simulink model "model"  (R2014a)
(part 2 of 3)

  _CN_171253574_150000_CN_129055610_150000 : powerlib/Elements/Distributed Parameters Line  Phases=3  Frequency=60  Resistance=[0.01273 0.3864]  Inductance="[0.9337e-3  4.1264e-3]"  Capacitance=[12.74e-9 7.751e-9]  Length=23.0398  x1=[0 0 0 0; 0.0001244 0 0 0; 0.0002488 0 0 0; 0.0003733 0 0 0; 0.0004977 0 0 0; 0.0006221 0 0 0]  x2=[0 0 0 0; 0.0001244 0 0 0; 0.0002488 0 0 0; 0.0003733 0 0 0; 0.0004977 0 0 0; 0.0006221 0 0 0]  x3=[0 0 0 0; 0.0001244 0 0 0; 0.0002488 0 0 0; 0.0003733 0 0 0; 0.0004977 0 0 0; 0.0006221 0 0 0]  x4=[0 0 0 0; 0.0001244 0 0 0; 0.0002488 0 0 0; 0.0003733 0 0 0; 0.0004977 0 0 0; 0.0006221 0 0 0]  x5=0  V1=ones(3,3)  V2=ones(3,3)  I1=ones(3,3)  I2=ones(3,3)  nHarmo=1  Measurements=None
  _CN_171253574_150000_CN_163226993_150000 : powerlib/Elements/Distributed Parameters Line  Phases=3  Frequency=60  Resistance=[0.01273 0.3864]  Inductance="[0.9337e-3  4.1264e-3]"  Capacitance=[12.74e-9 7.751e-9]  Length=4.3634  x1=[0 0 0 0; 0.0001244 0 0 0; 0.0002488 0 0 0; 0.0003733 0 0 0; 0.0004977 0 0 0; 0.0006221 0 0 0]  x2=[0 0 0 0; 0.0001244 0 0 0; 0.0002488 0 0 0; 0.0003733 0 0 0; 0.0004977 0 0 0; 0.0006221 0 0 0]  x3=[0 0 0 0; 0.0001244 0 0 0; 0.0002488 0 0 0; 0.0003733 0 0 0; 0.0004977 0 0 0; 0.0006221 0 0 0]  x4=[0 0 0 0; 0.0001244 0 0 0; 0.0002488 0 0 0; 0.0003733 0 0 0; 0.0004977 0 0 0; 0.0006221 0 0 0]  x5=0  V1=ones(3,3)  V2=ones(3,3)  I1=ones(3,3)  I2=ones(3,3)  nHarmo=1  Measurements=None
  _CN_183668286_220000_CN_151168335_220000 : powerlib/Elements/Distributed Parameters Line  Phases=3  Frequency=60  Resistance=[0.01273 0.3864]  Inductance="[0.9337e-3  4.1264e-3]"  Capacitance=[12.74e-9 7.751e-9]  Length=7.5354  x1=[0 0 0 0; 0.0001244 0 0 0; 0.0002488 0 0 0; 0.0003733 0 0 0; 0.0004977 0 0 0; 0.0006221 0 0 0]  x2=[0 0 0 0; 0.0001244 0 0 0; 0.0002488 0 0 0; 0.0003733 0 0 0; 0.0004977 0 0 0; 0.0006221 0 0 0]  x3=[0 0 0 0; 0.0001244 0 0 0; 0.0002488 0 0 0; 0.0003733 0 0 0; 0.0004977 0 0 0; 0.0006221 0 0 0]  x4=[0 0 0 0; 0.0001244 0 0 0; 0.0002488 0 0 0; 0.0003733 0 0 0; 0.0004977 0 0 0; 0.0006221 0 0 0]  x5=0  V1=ones(3,3)  V2=ones(3,3)  I1=ones(3,3)  I2=ones(3,3)  nHarmo=1  Measurements=None
  _CN_24636044_150000_CN_402947133_150000 : powerlib/Elements/Distributed Parameters Line  Phases=3  Frequency=60  Resistance=[0.01273 0.3864]  Inductance="[0.9337e-3  4.1264e-3]"  Capacitance=[12.74e-9 7.751e-9]  Length=13.2604  x1=[0 0 0 0; 0.0001244 0 0 0; 0.0002488 0 0 0; 0.0003733 0 0 0; 0.0004977 0 0 0; 0.0006221 0 0 0]  x2=[0 0 0 0; 0.0001244 0 0 0; 0.0002488 0 0 0; 0.0003733 0 0 0; 0.0004977 0 0 0; 0.0006221 0 0 0]  x3=[0 0 0 0; 0.0001244 0 0 0; 0.0002488 0 0 0; 0.0003733 0 0 0; 0.0004977 0 0 0; 0.0006221 0 0 0]  x4=[0 0 0 0; 0.0001244 0 0 0; 0.0002488 0 0 0; 0.0003733 0 0 0; 0.0004977 0 0 0; 0.0006221 0 0 0]  x5=0  V1=ones(3,3)  V2=ones(3,3)  I1=ones(3,3)  I2=ones(3,3)  nHarmo=1  Measurements=None
  _CN_24636044_220000_CN_131715746_220000 : powerlib/Elements/Distributed Parameters Line  Phases=3  Frequency=60  Resistance=[0.01273 0.3864]  Inductance="[0.9337e-3  4.1264e-3]"  Capacitance=[12.74e-9 7.751e-9]  Length=90.51  x1=[0 0 0 0; 0.0001244 0 0 0; 0.0002488 0 0 0; 0.0003733 0 0 0; 0.0004977 0 0 0; 0.0006221 0 0 0]  x2=[0 0 0 0; 0.0001244 0 0 0; 0.0002488 0 0 0; 0.0003733 0 0 0; 0.0004977 0 0 0; 0.0006221 0 0 0]  x3=[0 0 0 0; 0.0001244 0 0 0; 0.0002488 0 0 0; 0.0003733 0 0 0; 0.0004977 0 0 0; 0.0006221 0 0 0]  x4=[0 0 0 0; 0.0001244 0 0 0; 0.0002488 0 0 0; 0.0003733 0 0 0; 0.0004977 0 0 0; 0.0006221 0 0 0]  x5=0  V1=ones(3,3)  V2=ones(3,3)  I1=ones(3,3)  I2=ones(3,3)  nHarmo=1  Measurements=None
  _CN_24636044_220000_CN_144651478_220000 : powerlib/Elements/Distributed Parameters Line  Phases=3  Frequency=60  Resistance=[0.01273 0.3864]  Inductance="[0.9337e-3  4.1264e-3]"  Capacitance=[12.74e-9 7.751e-9]  Length=28.1072  x1=[0 0 0 0; 0.0001244 0 0 0; 0.0002488 0 0 0; 0.0003733 0 0 0; 0.0004977 0 0 0; 0.0006221 0 0 0]  x2=[0 0 0 0; 0.0001244 0 0 0; 0.0002488 0 0 0; 0.0003733 0 0 0; 0.0004977 0 0 0; 0.0006221 0 0 0]  x3=[0 0 0 0; 0.0001244 0 0 0; 0.0002488 0 0 0; 0.0003733 0 0 0; 0.0004977 0 0 0; 0.0006221 0 0 0]  x4=[0 0 0 0; 0.0001244 0 0 0; 0.0002488 0 0 0; 0.0003733 0 0 0; 0.0004977 0 0 0; 0.0006221 0 0 0]  x5=0  V1=ones(3,3)  V2=ones(3,3)  I1=ones(3,3)  I2=ones(3,3)  nHarmo=1  Measurements=None
  _CN_24636044_220000_CN_144654759_220000 : powerlib/Elements/Distributed Parameters Line  Phases=3  Frequency=60  Resistance=[0.01273 0.3864]  Inductance="[0.9337e-3  4.1264e-3]"  Capacitance=[12.74e-9 7.751e-9]  Length=18.5067  x1=[0 0 0 0; 0.0001244 0 0 0; 0.0002488 0 0 0; 0.0003733 0 0 0; 0.0004977 0 0 0; 0.0006221 0 0 0]  x2=[0 0 0 0; 0.0001244 0 0 0; 0.0002488 0 0 0; 0.0003733 0 0 0; 0.0004977 0 0 0; 0.0006221 0 0 0]  x3=[0 0 0 0; 0.0001244 0 0 0; 0.0002488 0 0 0; 0.0003733 0 0 0; 0.0004977 0 0 0; 0.0006221 0 0 0]  x4=[0 0 0 0; 0.0001244 0 0 0; 0.0002488 0 0 0; 0.0003733 0 0 0; 0.0004977 0 0 0; 0.0006221 0 0 0]  x5=0  V1=ones(3,3)  V2=ones(3,3)  I1=ones(3,3)  I2=ones(3,3)  nHarmo=1  Measurements=None
  _CN_24636044_220000_CN_144762180_220000 : powerlib/Elements/Distributed Parameters Line  Phases=3  Frequency=60  Resistance=[0.01273 0.3864]  Inductance="[0.9337e-3  4.1264e-3]"  Capacitance=[12.74e-9 7.751e-9]  Length=13.8029  x1=[0 0 0 0; 0.0001244 0 0 0; 0.0002488 0 0 0; 0.0003733 0 0 0; 0.0004977 0 0 0; 0.0006221 0 0 0]  x2=[0 0 0 0; 0.0001244 0 0 0; 0.0002488 0 0 0; 0.0003733 0 0 0; 0.0004977 0 0 0; 0.0006221 0 0 0]  x3=[0 0 0 0; 0.0001244 0 0 0; 0.0002488 0 0 0; 0.0003733 0 0 0; 0.0004977 0 0 0; 0.0006221 0 0 0]  x4=[0 0 0 0; 0.0001244 0 0 0; 0.0002488 0 0 0; 0.0003733 0 0 0; 0.0004977 0 0 0; 0.0006221 0 0 0]  x5=0  V1=ones(3,3)  V2=ones(3,3)  I1=ones(3,3)  I2=ones(3,3)  nHarmo=1  Measurements=None
  _CN_24636044_220000_CN_151166980_220000 : powerlib/Elements/Distributed Parameters Line  Phases=3  Frequency=60  Resistance=[0.01273 0.3864]  Inductance="[0.9337e-3  4.1264e-3]"  Capacitance=[12.74e-9 7.751e-9]  Length=57.0251  x1=[0 0 0 0; 0.0001244 0 0 0; 0.0002488 0 0 0; 0.0003733 0 0 0; 0.0004977 0 0 0; 0.0006221 0 0 0]  x2=[0 0 0 0; 0.0001244 0 0 0; 0.0002488 0 0 0; 0.0003733 0 0 0; 0.0004977 0 0 0; 0.0006221 0 0 0]  x3=[0 0 0 0; 0.0001244 0 0 0; 0.0002488 0 0 0; 0.0003733 0 0 0; 0.0004977 0 0 0; 0.0006221 0 0 0]  x4=[0 0 0 0; 0.0001244 0 0 0; 0.0002488 0 0 0; 0.0003733 0 0 0; 0.0004977 0 0 0; 0.0006221 0 0 0]  x5=0  V1=ones(3,3)  V2=ones(3,3)  I1=ones(3,3)  I2=ones(3,3)  nHarmo=1  Measurements=None
  _CN_24636044_220000_CN_151168335_220000 : powerlib/Elements/Distributed Parameters Line  Phases=3  Frequency=60  Resistance=[0.01273 0.3864]  Inductance="[0.9337e-3  4.1264e-3]"  Capacitance=[12.74e-9 7.751e-9]  Length=19.5147  x1=[0 0 0 0; 0.0001244 0 0 0; 0.0002488 0 0 0; 0.0003733 0 0 0; 0.0004977 0 0 0; 0.0006221 0 0 0]  x2=[0 0 0 0; 0.0001244 0 0 0; 0.0002488 0 0 0; 0.0003733 0 0 0; 0.0004977 0 0 0; 0.0006221 0 0 0]  x3=[0 0 0 0; 0.0001244 0 0 0; 0.0002488 0 0 0; 0.0003733 0 0 0; 0.0004977 0 0 0; 0.0006221 0 0 0]  x4=[0 0 0 0; 0.0001244 0 0 0; 0.0002488 0 0 0; 0.0003733 0 0 0; 0.0004977 0 0 0; 0.0006221 0 0 0]  x5=0  V1=ones(3,3)  V2=ones(3,3)  I1=ones(3,3)  I2=ones(3,3)  nHarmo=1  Measurements=None
  _CN_24636044_220000_CN_24636062_220000 : powerlib/Elements/Distributed Parameters Line  Phases=3  Frequency=60  Resistance=[0.01273 0.3864]  Inductance="[0.9337e-3  4.1264e-3]"  Capacitance=[12.74e-9 7.751e-9]  Length=15.5637  x1=[0 0 0 0; 0.0001244 0 0 0; 0.0002488 0 0 0; 0.0003733 0 0 0; 0.0004977 0 0 0; 0.0006221 0 0 0]  x2=[0 0 0 0; 0.0001244 0 0 0; 0.0002488 0 0 0; 0.0003733 0 0 0; 0.0004977 0 0 0; 0.0006221 0 0 0]  x3=[0 0 0 0; 0.0001244 0 0 0; 0.0002488 0 0 0; 0.0003733 0 0 0; 0.0004977 0 0 0; 0.0006221 0 0 0]  x4=[0 0 0 0; 0.0001244 0 0 0; 0.0002488 0 0 0; 0.0003733 0 0 0; 0.0004977 0 0 0; 0.0006221 0 0 0]  x5=0  V1=ones(3,3)  V2=ones(3,3)  I1=ones(3,3)  I2=ones(3,3)  nHarmo=1  Measurements=None
  _CN_24636044_220000_CN_435865807_220000 : powerlib/Elements/Distributed Parameters Line  Phases=3  Frequency=60  Resistance=[0.01273 0.3864]  Inductance="[0.9337e-3  4.1264e-3]"  Capacitance=[12.74e-9 7.751e-9]  Length=24.8935  x1=[0 0 0 0; 0.0001244 0 0 0; 0.0002488 0 0 0; 0.0003733 0 0 0; 0.0004977 0 0 0; 0.0006221 0 0 0]  x2=[0 0 0 0; 0.0001244 0 0 0; 0.0002488 0 0 0; 0.0003733 0 0 0; 0.0004977 0 0 0; 0.0006221 0 0 0]  x3=[0 0 0 0; 0.0001244 0 0 0; 0.0002488 0 0 0; 0.0003733 0 0 0; 0.0004977 0 0 0; 0.0006221 0 0 0]  x4=[0 0 0 0; 0.0001244 0 0 0; 0.0002488 0 0 0; 0.0003733 0 0 0; 0.0004977 0 0 0; 0.0006221 0 0 0]  x5=0  V1=ones(3,3)  V2=ones(3,3)  I1=ones(3,3)  I2=ones(3,3)  nHarmo=1  Measurements=None
  _CN_24636044_400000_CN_129055610_400000 : powerlib/Elements/Distributed Parameters Line  Phases=3  Frequency=60  Resistance=[0.01273 0.3864]  Inductance="[0.9337e-3  4.1264e-3]"  Capacitance=[12.74e-9 7.751e-9]  Length=68.1978  x1=[0 0 0 0; 0.0001244 0 0 0; 0.0002488 0 0 0; 0.0003733 0 0 0; 0.0004977 0 0 0; 0.0006221 0 0 0]  x2=[0 0 0 0; 0.0001244 0 0 0; 0.0002488 0 0 0; 0.0003733 0 0 0; 0.0004977 0 0 0; 0.0006221 0 0 0]  x3=[0 0 0 0; 0.0001244 0 0 0; 0.0002488 0 0 0; 0.0003733 0 0 0; 0.0004977 0 0 0; 0.0006221 0 0 0]  x4=[0 0 0 0; 0.0001244 0 0 0; 0.0002488 0 0 0; 0.0003733 0 0 0; 0.0004977 0 0 0; 0.0006221 0 0 0]  x5=0  V1=ones(3,3)  V2=ones(3,3)  I1=ones(3,3)  I2=ones(3,3)  nHarmo=1  Measurements=None
  _CN_24636044_400000_CN_131715746_400000 : powerlib/Elements/Distributed Parameters Line  Phases=3  Frequency=60  Resistance=[0.01273 0.3864]  Inductance="[0.9337e-3  4.1264e-3]"  Capacitance=[12.74e-9 7.751e-9]  Length=53.1895  x1=[0 0 0 0; 0.0001244 0 0 0; 0.0002488 0 0 0; 0.0003733 0 0 0; 0.0004977 0 0 0; 0.0006221 0 0 0]  x2=[0 0 0 0; 0.0001244 0 0 0; 0.0002488 0 0 0; 0.0003733 0 0 0; 0.0004977 0 0 0; 0.0006221 0 0 0]  x3=[0 0 0 0; 0.0001244 0 0 0; 0.0002488 0 0 0; 0.0003733 0 0 0; 0.0004977 0 0 0; 0.0006221 0 0 0]  x4=[0 0 0 0; 0.0001244 0 0 0; 0.0002488 0 0 0; 0.0003733 0 0 0; 0.0004977 0 0 0; 0.0006221 0 0 0]  x5=0  V1=ones(3,3)  V2=ones(3,3)  I1=ones(3,3)  I2=ones(3,3)  nHarmo=1  Measurements=None
  _CN_24636044_400000_CN_144608818_400000 : powerlib/Elements/Distributed Parameters Line  Phases=3  Frequency=60  Resistance=[0.01273 0.3864]  Inductance="[0.9337e-3  4.1264e-3]"  Capacitance=[12.74e-9 7.751e-9]  Length=25.0456  x1=[0 0 0 0; 0.0001244 0 0 0; 0.0002488 0 0 0; 0.0003733 0 0 0; 0.0004977 0 0 0; 0.0006221 0 0 0]  x2=[0 0 0 0; 0.0001244 0 0 0; 0.0002488 0 0 0; 0.0003733 0 0 0; 0.0004977 0 0 0; 0.0006221 0 0 0]  x3=[0 0 0 0; 0.0001244 0 0 0; 0.0002488 0 0 0; 0.0003733 0 0 0; 0.0004977 0 0 0; 0.0006221 0 0 0]  x4=[0 0 0 0; 0.0001244 0 0 0; 0.0002488 0 0 0; 0.0003733 0 0 0; 0.0004977 0 0 0; 0.0006221 0 0 0]  x5=0  V1=ones(3,3)  V2=ones(3,3)  I1=ones(3,3)  I2=ones(3,3)  nHarmo=1  Measurements=None
  _CN_24636044_400000_CN_151168335_400000 : powerlib/Elements/Distributed Parameters Line  Phases=3  Frequency=60  Resistance=[0.01273 0.3864]  Inductance="[0.9337e-3  4.1264e-3]"  Capacitance=[12.74e-9 7.751e-9]  Length=18.3774  x1=[0 0 0 0; 0.0001244 0 0 0; 0.0002488 0 0 0; 0.0003733 0 0 0; 0.0004977 0 0 0; 0.0006221 0 0 0]  x2=[0 0 0 0; 0.0001244 0 0 0; 0.0002488 0 0 0; 0.0003733 0 0 0; 0.0004977 0 0 0; 0.0006221 0 0 0]  x3=[0 0 0 0; 0.0001244 0 0 0; 0.0002488 0 0 0; 0.0003733 0 0 0; 0.0004977 0 0 0; 0.0006221 0 0 0]  x4=[0 0 0 0; 0.0001244 0 0 0; 0.0002488 0 0 0; 0.0003733 0 0 0; 0.0004977 0 0 0; 0.0006221 0 0 0]  x5=0  V1=ones(3,3)  V2=ones(3,3)  I1=ones(3,3)  I2=ones(3,3)  nHarmo=1  Measurements=None
  _CN_24636062_220000_CN_183668286_220000 : powerlib/Elements/Distributed Parameters Line  Phases=3  Frequency=60  Resistance=[0.01273 0.3864]  Inductance="[0.9337e-3  4.1264e-3]"  Capacitance=[12.74e-9 7.751e-9]  Length=4.494  x1=[0 0 0 0; 0.0001244 0 0 0; 0.0002488 0 0 0; 0.0003733 0 0 0; 0.0004977 0 0 0; 0.0006221 0 0 0]  x2=[0 0 0 0; 0.0001244 0 0 0; 0.0002488 0 0 0; 0.0003733 0 0 0; 0.0004977 0 0 0; 0.0006221 0 0 0]  x3=[0 0 0 0; 0.0001244 0 0 0; 0.0002488 0 0 0; 0.0003733 0 0 0; 0.0004977 0 0 0; 0.0006221 0 0 0]  x4=[0 0 0 0; 0.0001244 0 0 0; 0.0002488 0 0 0; 0.0003733 0 0 0; 0.0004977 0 0 0; 0.0006221 0 0 0]  x5=0  V1=ones(3,3)  V2=ones(3,3)  I1=ones(3,3)  I2=ones(3,3)  nHarmo=1  Measurements=None
  _CN_402947133_220000_CN_144762180_220000 : powerlib/Elements/Distributed Parameters Line  Phases=3  Frequency=60  Resistance=[0.01273 0.3864]  Inductance="[0.9337e-3  4.1264e-3]"  Capacitance=[12.74e-9 7.751e-9]  Length=1.5227  x1=[0 0 0 0; 0.0001244 0 0 0; 0.0002488 0 0 0; 0.0003733 0 0 0; 0.0004977 0 0 0; 0.0006221 0 0 0]  x2=[0 0 0 0; 0.0001244 0 0 0; 0.0002488 0 0 0; 0.0003733 0 0 0; 0.0004977 0 0 0; 0.0006221 0 0 0]  x3=[0 0 0 0; 0.0001244 0 0 0; 0.0002488 0 0 0; 0.0003733 0 0 0; 0.0004977 0 0 0; 0.0006221 0 0 0]  x4=[0 0 0 0; 0.0001244 0 0 0; 0.0002488 0 0 0; 0.0003733 0 0 0; 0.0004977 0 0 0; 0.0006221 0 0 0]  x5=0  V1=ones(3,3)  V2=ones(3,3)  I1=ones(3,3)  I2=ones(3,3)  nHarmo=1  Measurements=None
  _CN_435865807_220000_CN_131715746_220000 : powerlib/Elements/Distributed Parameters Line  Phases=3  Frequency=60  Resistance=[0.01273 0.3864]  Inductance="[0.9337e-3  4.1264e-3]"  Capacitance=[12.74e-9 7.751e-9]  Length=38.8013  x1=[0 0 0 0; 0.0001244 0 0 0; 0.0002488 0 0 0; 0.0003733 0 0 0; 0.0004977 0 0 0; 0.0006221 0 0 0]  x2=[0 0 0 0; 0.0001244 0 0 0; 0.0002488 0 0 0; 0.0003733 0 0 0; 0.0004977 0 0 0; 0.0006221 0 0 0]  x3=[0 0 0 0; 0.0001244 0 0 0; 0.0002488 0 0 0; 0.0003733 0 0 0; 0.0004977 0 0 0; 0.0006221 0 0 0]  x4=[0 0 0 0; 0.0001244 0 0 0; 0.0002488 0 0 0; 0.0003733 0 0 0; 0.0004977 0 0 0; 0.0006221 0 0 0]  x5=0  V1=ones(3,3)  V2=ones(3,3)  I1=ones(3,3)  I2=ones(3,3)  nHarmo=1  Measurements=None
  _CN_435865807_220000_CN_144596347_220000 : powerlib/Elements/Distributed Parameters Line  Phases=3  Frequency=60  Resistance=[0.01273 0.3864]  Inductance="[0.9337e-3  4.1264e-3]"  Capacitance=[12.74e-9 7.751e-9]  Length=34.808  x1=[0 0 0 0; 0.0001244 0 0 0; 0.0002488 0 0 0; 0.0003733 0 0 0; 0.0004977 0 0 0; 0.0006221 0 0 0]  x2=[0 0 0 0; 0.0001244 0 0 0; 0.0002488 0 0 0; 0.0003733 0 0 0; 0.0004977 0 0 0; 0.0006221 0 0 0]  x3=[0 0 0 0; 0.0001244 0 0 0; 0.0002488 0 0 0; 0.0003733 0 0 0; 0.0004977 0 0 0; 0.0006221 0 0 0]  x4=[0 0 0 0; 0.0001244 0 0 0; 0.0002488 0 0 0; 0.0003733 0 0 0; 0.0004977 0 0 0; 0.0006221 0 0 0]  x5=0  V1=ones(3,3)  V2=ones(3,3)  I1=ones(3,3)  I2=ones(3,3)  nHarmo=1  Measurements=None
  _CN_435865807_220000_CN_144703168_220000 : powerlib/Elements/Distributed Parameters Line  Phases=3  Frequency=60  Resistance=[0.01273 0.3864]  Inductance="[0.9337e-3  4.1264e-3]"  Capacitance=[12.74e-9 7.751e-9]  Length=56.7538  x1=[0 0 0 0; 0.0001244 0 0 0; 0.0002488 0 0 0; 0.0003733 0 0 0; 0.0004977 0 0 0; 0.0006221 0 0 0]  x2=[0 0 0 0; 0.0001244 0 0 0; 0.0002488 0 0 0; 0.0003733 0 0 0; 0.0004977 0 0 0; 0.0006221 0 0 0]  x3=[0 0 0 0; 0.0001244 0 0 0; 0.0002488 0 0 0; 0.0003733 0 0 0; 0.0004977 0 0 0; 0.0006221 0 0 0]  x4=[0 0 0 0; 0.0001244 0 0 0; 0.0002488 0 0 0; 0.0003733 0 0 0; 0.0004977 0 0 0; 0.0006221 0 0 0]  x5=0  V1=ones(3,3)  V2=ones(3,3)  I1=ones(3,3)  I2=ones(3,3)  nHarmo=1  Measurements=None
  _CN_47895778_220000_CN_127205502_220000 : powerlib/Elements/Distributed Parameters Line  Phases=3  Frequency=60  Resistance=[0.01273 0.3864]  Inductance="[0.9337e-3  4.1264e-3]"  Capacitance=[12.74e-9 7.751e-9]  Length=41.7466  x1=[0 0 0 0; 0.0001244 0 0 0; 0.0002488 0 0 0; 0.0003733 0 0 0; 0.0004977 0 0 0; 0.0006221 0 0 0]  x2=[0 0 0 0; 0.0001244 0 0 0; 0.0002488 0 0 0; 0.0003733 0 0 0; 0.0004977 0 0 0; 0.0006221 0 0 0]  x3=[0 0 0 0; 0.0001244 0 0 0; 0.0002488 0 0 0; 0.0003733 0 0 0; 0.0004977 0 0 0; 0.0006221 0 0 0]  x4=[0 0 0 0; 0.0001244 0 0 0; 0.0002488 0 0 0; 0.0003733 0 0 0; 0.0004977 0 0 0; 0.0006221 0 0 0]  x5=0  V1=ones(3,3)  V2=ones(3,3)  I1=ones(3,3)  I2=ones(3,3)  nHarmo=1  Measurements=None
  _CN_47911346_220000_CN_47895778_220000 : powerlib/Elements/Distributed Parameters Line  Phases=3  Frequency=60  Resistance=[0.01273 0.3864]  Inductance="[0.9337e-3  4.1264e-3]"  Capacitance=[12.74e-9 7.751e-9]  Length=0.71591  x1=[0 0 0 0; 0.0001244 0 0 0; 0.0002488 0 0 0; 0.0003733 0 0 0; 0.0004977 0 0 0; 0.0006221 0 0 0]  x2=[0 0 0 0; 0.0001244 0 0 0; 0.0002488 0 0 0; 0.0003733 0 0 0; 0.0004977 0 0 0; 0.0006221 0 0 0]  x3=[0 0 0 0; 0.0001244 0 0 0; 0.0002488 0 0 0; 0.0003733 0 0 0; 0.0004977 0 0 0; 0.0006221 0 0 0]  x4=[0 0 0 0; 0.0001244 0 0 0; 0.0002488 0 0 0; 0.0003733 0 0 0; 0.0004977 0 0 0; 0.0006221 0 0 0]  x5=0  V1=ones(3,3)  V2=ones(3,3)  I1=ones(3,3)  I2=ones(3,3)  nHarmo=1  Measurements=None
  _CN_47911346_400000_CN_144327157_400000 : powerlib/Elements/Distributed Parameters Line  Phases=3  Frequency=60  Resistance=[0.01273 0.3864]  Inductance="[0.9337e-3  4.1264e-3]"  Capacitance=[12.74e-9 7.751e-9]  Length=17.6368  x1=[0 0 0 0; 0.0001244 0 0 0; 0.0002488 0 0 0; 0.0003733 0 0 0; 0.0004977 0 0 0; 0.0006221 0 0 0]  x2=[0 0 0 0; 0.0001244 0 0 0; 0.0002488 0 0 0; 0.0003733 0 0 0; 0.0004977 0 0 0; 0.0006221 0 0 0]  x3=[0 0 0 0; 0.0001244 0 0 0; 0.0002488 0 0 0; 0.0003733 0 0 0; 0.0004977 0 0 0; 0.0006221 0 0 0]  x4=[0 0 0 0; 0.0001244 0 0 0; 0.0002488 0 0 0; 0.0003733 0 0 0; 0.0004977 0 0 0; 0.0006221 0 0 0]  x5=0  V1=ones(3,3)  V2=ones(3,3)  I1=ones(3,3)  I2=ones(3,3)  nHarmo=1  Measurements=None
  bus1 : powerlib/Measurements/Load Flow Bus  LConnTagsString=a  ID=bus1  Vbase=150000  Vref=1  Vangle=0  VLF=1  angleLF=0
      settings: AttributesFormatString=|
      | %<ID>
      | %<Vbase>V
      | %<VLF>pu
      | %<angleLF>deg.
      | %<Name>
  bus10 : powerlib/Measurements/Load Flow Bus  LConnTagsString=a  ID=bus10  Vbase=150000  Vref=1  Vangle=0  VLF=1  angleLF=0
      settings: AttributesFormatString=|
      | %<ID>
      | %<Vbase>V
      | %<VLF>pu
      | %<angleLF>deg.
      | %<Name>
  bus100 : powerlib/Measurements/Load Flow Bus  LConnTagsString=a  ID=bus100  Vbase=400000  Vref=1  Vangle=0  VLF=1  angleLF=0
      settings: AttributesFormatString=|
      | %<ID>
      | %<Vbase>V
      | %<VLF>pu
      | %<angleLF>deg.
      | %<Name>
  bus101 : powerlib/Measurements/Load Flow Bus  LConnTagsString=a  ID=bus101  Vbase=400000  Vref=1  Vangle=0  VLF=1  angleLF=0
      settings: AttributesFormatString=|
      | %<ID>
      | %<Vbase>V
      | %<VLF>pu
      | %<angleLF>deg.
      | %<Name>
  bus102 : powerlib/Measurements/Load Flow Bus  LConnTagsString=a  ID=bus102  Vbase=400000  Vref=1  Vangle=0  VLF=1  angleLF=0
      settings: AttributesFormatString=|
      | %<ID>
      | %<Vbase>V
      | %<VLF>pu
      | %<angleLF>deg.
      | %<Name>
  bus103 : powerlib/Measurements/Load Flow Bus  LConnTagsString=a  ID=bus103  Vbase=400000  Vref=1  Vangle=0  VLF=1  angleLF=0
      settings: AttributesFormatString=|
      | %<ID>
      | %<Vbase>V
      | %<VLF>pu
      | %<angleLF>deg.
      | %<Name>
  bus104 : powerlib/Measurements/Load Flow Bus  LConnTagsString=a  ID=bus104  Vbase=400000  Vref=1  Vangle=0  VLF=1  angleLF=0
      settings: AttributesFormatString=|
      | %<ID>
      | %<Vbase>V
      | %<VLF>pu
      | %<angleLF>deg.
      | %<Name>
  bus105 : powerlib/Measurements/Load Flow Bus  LConnTagsString=a  ID=bus105  Vbase=400000  Vref=1  Vangle=0  VLF=1  angleLF=0
      settings: AttributesFormatString=|
      | %<ID>
      | %<Vbase>V
      | %<VLF>pu
      | %<angleLF>deg.
      | %<Name>
  bus106 : powerlib/Measurements/Load Flow Bus  LConnTagsString=a  ID=bus106  Vbase=400000  Vref=1  Vangle=0  VLF=1  angleLF=0
      settings: AttributesFormatString=|
      | %<ID>
      | %<Vbase>V
      | %<VLF>pu
      | %<angleLF>deg.
      | %<Name>
  bus107 : powerlib/Measurements/Load Flow Bus  LConnTagsString=a  ID=bus107  Vbase=400000  Vref=1  Vangle=0  VLF=1  angleLF=0
      settings: AttributesFormatString=|
      | %<ID>
      | %<Vbase>V
      | %<VLF>pu
      | %<angleLF>deg.
      | %<Name>
  bus108 : powerlib/Measurements/Load Flow Bus  LConnTagsString=a  ID=bus108  Vbase=400000  Vref=1  Vangle=0  VLF=1  angleLF=0
      settings: AttributesFormatString=|
      | %<ID>
      | %<Vbase>V
      | %<VLF>pu
      | %<angleLF>deg.
      | %<Name>
  bus109 : powerlib/Measurements/Load Flow Bus  LConnTagsString=a  ID=bus109  Vbase=400000  Vref=1  Vangle=0  VLF=1  angleLF=0
      settings: AttributesFormatString=|
      | %<ID>
      | %<Vbase>V
      | %<VLF>pu
      | %<angleLF>deg.
      | %<Name>
  bus11 : powerlib/Measurements/Load Flow Bus  LConnTagsString=a  ID=bus11  Vbase=150000  Vref=1  Vangle=0  VLF=1  angleLF=0
      settings: AttributesFormatString=|
      | %<ID>
      | %<Vbase>V
      | %<VLF>pu
      | %<angleLF>deg.
      | %<Name>
  bus110 : powerlib/Measurements/Load Flow Bus  LConnTagsString=a  ID=bus110  Vbase=400000  Vref=1  Vangle=0  VLF=1  angleLF=0
      settings: AttributesFormatString=|
      | %<ID>
      | %<Vbase>V
      | %<VLF>pu
      | %<angleLF>deg.
      | %<Name>
  bus111 : powerlib/Measurements/Load Flow Bus  LConnTagsString=a  ID=bus111  Vbase=400000  Vref=1  Vangle=0  VLF=1  angleLF=0
      settings: AttributesFormatString=|
      | %<ID>
      | %<Vbase>V
      | %<VLF>pu
      | %<angleLF>deg.
      | %<Name>
  bus112 : powerlib/Measurements/Load Flow Bus  LConnTagsString=a  ID=bus112  Vbase=400000  Vref=1  Vangle=0  VLF=1  angleLF=0
      settings: AttributesFormatString=|
      | %<ID>
      | %<Vbase>V
      | %<VLF>pu
      | %<angleLF>deg.
      | %<Name>
  bus113 : powerlib/Measurements/Load Flow Bus  LConnTagsString=a  ID=bus113  Vbase=400000  Vref=1  Vangle=0  VLF=1  angleLF=0
      settings: AttributesFormatString=|
      | %<ID>
      | %<Vbase>V
      | %<VLF>pu
      | %<angleLF>deg.
      | %<Name>
  bus114 : powerlib/Measurements/Load Flow Bus  LConnTagsString=a  ID=bus114  Vbase=400000  Vref=1  Vangle=0  VLF=1  angleLF=0
      settings: AttributesFormatString=|
      | %<ID>
      | %<Vbase>V
      | %<VLF>pu
      | %<angleLF>deg.
      | %<Name>
  bus115 : powerlib/Measurements/Load Flow Bus  LConnTagsString=a  ID=bus115  Vbase=400000  Vref=1  Vangle=0  VLF=1  angleLF=0
      settings: AttributesFormatString=|
      | %<ID>
      | %<Vbase>V
      | %<VLF>pu
      | %<angleLF>deg.
      | %<Name>
  bus116 : powerlib/Measurements/Load Flow Bus  LConnTagsString=a  ID=bus116  Vbase=400000  Vref=1  Vangle=0  VLF=1  angleLF=0
      settings: AttributesFormatString=|
      | %<ID>
      | %<Vbase>V
      | %<VLF>pu
      | %<angleLF>deg.
      | %<Name>
  bus117 : powerlib/Measurements/Load Flow Bus  LConnTagsString=a  ID=bus117  Vbase=400000  Vref=1  Vangle=0  VLF=1  angleLF=0
      settings: AttributesFormatString=|
      | %<ID>
      | %<Vbase>V
      | %<VLF>pu
      | %<angleLF>deg.
      | %<Name>
  bus118 : powerlib/Measurements/Load Flow Bus  LConnTagsString=a  ID=bus118  Vbase=400000  Vref=1  Vangle=0  VLF=1  angleLF=0
      settings: AttributesFormatString=|
      | %<ID>
      | %<Vbase>V
      | %<VLF>pu
      | %<angleLF>deg.
      | %<Name>
  bus119 : powerlib/Measurements/Load Flow Bus  LConnTagsString=a  ID=bus119  Vbase=400000  Vref=1  Vangle=0  VLF=1  angleLF=0
      settings: AttributesFormatString=|
      | %<ID>
      | %<Vbase>V
      | %<VLF>pu
      | %<angleLF>deg.
      | %<Name>
  bus12 : powerlib/Measurements/Load Flow Bus  LConnTagsString=a  ID=bus12  Vbase=150000  Vref=1  Vangle=0  VLF=1  angleLF=0
      settings: AttributesFormatString=|
      | %<ID>
      | %<Vbase>V
      | %<VLF>pu
      | %<angleLF>deg.
      | %<Name>
  bus120 : powerlib/Measurements/Load Flow Bus  LConnTagsString=a  ID=bus120  Vbase=400000  Vref=1  Vangle=0  VLF=1  angleLF=0
      settings: AttributesFormatString=|
      | %<ID>
      | %<Vbase>V
      | %<VLF>pu
      | %<angleLF>deg.
      | %<Name>
  bus121 : powerlib/Measurements/Load Flow Bus  LConnTagsString=a  ID=bus121  Vbase=400000  Vref=1  Vangle=0  VLF=1  angleLF=0
      settings: AttributesFormatString=|
      | %<ID>
      | %<Vbase>V
      | %<VLF>pu
      | %<angleLF>deg.
      | %<Name>
  bus122 : powerlib/Measurements/Load Flow Bus  LConnTagsString=a  ID=bus122  Vbase=400000  Vref=1  Vangle=0  VLF=1  angleLF=0
      settings: AttributesFormatString=|
      | %<ID>
      | %<Vbase>V
      | %<VLF>pu
      | %<angleLF>deg.
      | %<Name>
  bus123 : powerlib/Measurements/Load Flow Bus  LConnTagsString=a  ID=bus123  Vbase=400000  Vref=1  Vangle=0  VLF=1  angleLF=0
      settings: AttributesFormatString=|
      | %<ID>
      | %<Vbase>V
      | %<VLF>pu
      | %<angleLF>deg.
      | %<Name>
  bus124 : powerlib/Measurements/Load Flow Bus  LConnTagsString=a  ID=bus124  Vbase=400000  Vref=1  Vangle=0  VLF=1  angleLF=0
      settings: AttributesFormatString=|
      | %<ID>
      | %<Vbase>V
      | %<VLF>pu
      | %<angleLF>deg.
      | %<Name>
  bus125 : powerlib/Measurements/Load Flow Bus  LConnTagsString=a  ID=bus125  Vbase=400000  Vref=1  Vangle=0  VLF=1  angleLF=0
      settings: AttributesFormatString=|
      | %<ID>
      | %<Vbase>V
      | %<VLF>pu
      | %<angleLF>deg.
      | %<Name>
  bus126 : powerlib/Measurements/Load Flow Bus  LConnTagsString=a  ID=bus126  Vbase=400000  Vref=1  Vangle=0  VLF=1  angleLF=0
      settings: AttributesFormatString=|
      | %<ID>
      | %<Vbase>V
      | %<VLF>pu
      | %<angleLF>deg.
      | %<Name>
  bus127 : powerlib/Measurements/Load Flow Bus  LConnTagsString=a  ID=bus127  Vbase=150000  Vref=1  Vangle=0  VLF=1  angleLF=0
      settings: AttributesFormatString=|
      | %<ID>
      | %<Vbase>V
      | %<VLF>pu
      | %<angleLF>deg.
      | %<Name>
  bus128 : powerlib/Measurements/Load Flow Bus  LConnTagsString=a  ID=bus128  Vbase=150000  Vref=1  Vangle=0  VLF=1  angleLF=0
      settings: AttributesFormatString=|
      | %<ID>
      | %<Vbase>V
      | %<VLF>pu
      | %<angleLF>deg.
      | %<Name>
  bus129 : powerlib/Measurements/Load Flow Bus  LConnTagsString=a  ID=bus129  Vbase=150000  Vref=1  Vangle=0  VLF=1  angleLF=0
      settings: AttributesFormatString=|
      | %<ID>
      | %<Vbase>V
      | %<VLF>pu
      | %<angleLF>deg.
      | %<Name>
  bus13 : powerlib/Measurements/Load Flow Bus  LConnTagsString=a  ID=bus13  Vbase=150000  Vref=1  Vangle=0  VLF=1  angleLF=0
      settings: AttributesFormatString=|
      | %<ID>
      | %<Vbase>V
      | %<VLF>pu
      | %<angleLF>deg.
      | %<Name>
  bus130 : powerlib/Measurements/Load Flow Bus  LConnTagsString=a  ID=bus130  Vbase=150000  Vref=1  Vangle=0  VLF=1  angleLF=0
      settings: AttributesFormatString=|
      | %<ID>
      | %<Vbase>V
      | %<VLF>pu
      | %<angleLF>deg.
      | %<Name>
  bus131 : powerlib/Measurements/Load Flow Bus  LConnTagsString=a  ID=bus131  Vbase=150000  Vref=1  Vangle=0  VLF=1  angleLF=0
      settings: AttributesFormatString=|
      | %<ID>
      | %<Vbase>V
      | %<VLF>pu
      | %<angleLF>deg.
      | %<Name>
  bus132 : powerlib/Measurements/Load Flow Bus  LConnTagsString=a  ID=bus132  Vbase=150000  Vref=1  Vangle=0  VLF=1  angleLF=0
      settings: AttributesFormatString=|
      | %<ID>
      | %<Vbase>V
      | %<VLF>pu
      | %<angleLF>deg.
      | %<Name>
  bus133 : powerlib/Measurements/Load Flow Bus  LConnTagsString=a  ID=bus133  Vbase=150000  Vref=1  Vangle=0  VLF=1  angleLF=0
      settings: AttributesFormatString=|
      | %<ID>
      | %<Vbase>V
      | %<VLF>pu
      | %<angleLF>deg.
      | %<Name>
  bus134 : powerlib/Measurements/Load Flow Bus  LConnTagsString=a  ID=bus134  Vbase=150000  Vref=1  Vangle=0  VLF=1  angleLF=0
      settings: AttributesFormatString=|
      | %<ID>
      | %<Vbase>V
      | %<VLF>pu
      | %<angleLF>deg.
      | %<Name>
  bus135 : powerlib/Measurements/Load Flow Bus  LConnTagsString=a  ID=bus135  Vbase=150000  Vref=1  Vangle=0  VLF=1  angleLF=0
      settings: AttributesFormatString=|
      | %<ID>
      | %<Vbase>V
      | %<VLF>pu
      | %<angleLF>deg.
      | %<Name>
  bus136 : powerlib/Measurements/Load Flow Bus  LConnTagsString=a  ID=bus136  Vbase=150000  Vref=1  Vangle=0  VLF=1  angleLF=0
      settings: AttributesFormatString=|
      | %<ID>
      | %<Vbase>V
      | %<VLF>pu
      | %<angleLF>deg.
      | %<Name>
  bus137 : powerlib/Measurements/Load Flow Bus  LConnTagsString=a  ID=bus137  Vbase=150000  Vref=1  Vangle=0  VLF=1  angleLF=0
      settings: AttributesFormatString=|
      | %<ID>
      | %<Vbase>V
      | %<VLF>pu
      | %<angleLF>deg.
      | %<Name>
  bus138 : powerlib/Measurements/Load Flow Bus  LConnTagsString=a  ID=bus138  Vbase=150000  Vref=1  Vangle=0  VLF=1  angleLF=0
      settings: AttributesFormatString=|
      | %<ID>
      | %<Vbase>V
      | %<VLF>pu
      | %<angleLF>deg.
      | %<Name>
  bus139 : powerlib/Measurements/Load Flow Bus  LConnTagsString=a  ID=bus139  Vbase=150000  Vref=1  Vangle=0  VLF=1  angleLF=0
      settings: AttributesFormatString=|
      | %<ID>
      | %<Vbase>V
      | %<VLF>pu
      | %<angleLF>deg.
      | %<Name>
  bus14 : powerlib/Measurements/Load Flow Bus  LConnTagsString=a  ID=bus14  Vbase=150000  Vref=1  Vangle=0  VLF=1  angleLF=0
      settings: AttributesFormatString=|
      | %<ID>
      | %<Vbase>V
      | %<VLF>pu
      | %<angleLF>deg.
      | %<Name>
  bus140 : powerlib/Measurements/Load Flow Bus  LConnTagsString=a  ID=bus140  Vbase=150000  Vref=1  Vangle=0  VLF=1  angleLF=0
      settings: AttributesFormatString=|
      | %<ID>
      | %<Vbase>V
      | %<VLF>pu
      | %<angleLF>deg.
      | %<Name>
  bus141 : powerlib/Measurements/Load Flow Bus  LConnTagsString=a  ID=bus141  Vbase=150000  Vref=1  Vangle=0  VLF=1  angleLF=0
      settings: AttributesFormatString=|
      | %<ID>
      | %<Vbase>V
      | %<VLF>pu
      | %<angleLF>deg.
      | %<Name>
  bus142 : powerlib/Measurements/Load Flow Bus  LConnTagsString=a  ID=bus142  Vbase=150000  Vref=1  Vangle=0  VLF=1  angleLF=0
      settings: AttributesFormatString=|
      | %<ID>
      | %<Vbase>V
      | %<VLF>pu
      | %<angleLF>deg.
      | %<Name>
  bus143 : powerlib/Measurements/Load Flow Bus  LConnTagsString=a  ID=bus143  Vbase=150000  Vref=1  Vangle=0  VLF=1  angleLF=0
      settings: AttributesFormatString=|
      | %<ID>
      | %<Vbase>V
      | %<VLF>pu
      | %<angleLF>deg.
      | %<Name>
  bus144 : powerlib/Measurements/Load Flow Bus  LConnTagsString=a  ID=bus144  Vbase=150000  Vref=1  Vangle=0  VLF=1  angleLF=0
      settings: AttributesFormatString=|
      | %<ID>
      | %<Vbase>V
      | %<VLF>pu
      | %<angleLF>deg.
      | %<Name>
  bus145 : powerlib/Measurements/Load Flow Bus  LConnTagsString=a  ID=bus145  Vbase=150000  Vref=1  Vangle=0  VLF=1  angleLF=0
      settings: AttributesFormatString=|
      | %<ID>
      | %<Vbase>V
      | %<VLF>pu
      | %<angleLF>deg.
      | %<Name>
  bus146 : powerlib/Measurements/Load Flow Bus  LConnTagsString=a  ID=bus146  Vbase=150000  Vref=1  Vangle=0  VLF=1  angleLF=0
      settings: AttributesFormatString=|
      | %<ID>
      | %<Vbase>V
      | %<VLF>pu
      | %<angleLF>deg.
      | %<Name>
  bus147 : powerlib/Measurements/Load Flow Bus  LConnTagsString=a  ID=bus147  Vbase=150000  Vref=1  Vangle=0  VLF=1  angleLF=0
      settings: AttributesFormatString=|
      | %<ID>
      | %<Vbase>V
      | %<VLF>pu
      | %<angleLF>deg.
      | %<Name>
  bus148 : powerlib/Measurements/Load Flow Bus  LConnTagsString=a  ID=bus148  Vbase=150000  Vref=1  Vangle=0  VLF=1  angleLF=0
      settings: AttributesFormatString=|
      | %<ID>
      | %<Vbase>V
      | %<VLF>pu
      | %<angleLF>deg.
      | %<Name>
  bus149 : powerlib/Measurements/Load Flow Bus  LConnTagsString=a  ID=bus149  Vbase=150000  Vref=1  Vangle=0  VLF=1  angleLF=0
      settings: AttributesFormatString=|
      | %<ID>
      | %<Vbase>V
      | %<VLF>pu
      | %<angleLF>deg.
      | %<Name>
  bus15 : powerlib/Measurements/Load Flow Bus  LConnTagsString=a  ID=bus15  Vbase=150000  Vref=1  Vangle=0  VLF=1  angleLF=0
      settings: AttributesFormatString=|
      | %<ID>
      | %<Vbase>V
      | %<VLF>pu
      | %<angleLF>deg.
      | %<Name>
  bus150 : powerlib/Measurements/Load Flow Bus  LConnTagsString=a  ID=bus150  Vbase=150000  Vref=1  Vangle=0  VLF=1  angleLF=0
      settings: AttributesFormatString=|
      | %<ID>
      | %<Vbase>V
      | %<VLF>pu
      | %<angleLF>deg.
      | %<Name>
  bus151 : powerlib/Measurements/Load Flow Bus  LConnTagsString=a  ID=bus151  Vbase=150000  Vref=1  Vangle=0  VLF=1  angleLF=0
      settings: AttributesFormatString=|
      | %<ID>
      | %<Vbase>V
      | %<VLF>pu
      | %<angleLF>deg.
      | %<Name>
  bus152 : powerlib/Measurements/Load Flow Bus  LConnTagsString=a  ID=bus152  Vbase=150000  Vref=1  Vangle=0  VLF=1  angleLF=0
      settings: AttributesFormatString=|
      | %<ID>
      | %<Vbase>V
      | %<VLF>pu
      | %<angleLF>deg.
      | %<Name>
  bus153 : powerlib/Measurements/Load Flow Bus  LConnTagsString=a  ID=bus153  Vbase=150000  Vref=1  Vangle=0  VLF=1  angleLF=0
      settings: AttributesFormatString=|
      | %<ID>
      | %<Vbase>V
      | %<VLF>pu
      | %<angleLF>deg.
      | %<Name>
  bus154 : powerlib/Measurements/Load Flow Bus  LConnTagsString=a  ID=bus154  Vbase=150000  Vref=1  Vangle=0  VLF=1  angleLF=0
      settings: AttributesFormatString=|
      | %<ID>
      | %<Vbase>V
      | %<VLF>pu
      | %<angleLF>deg.
      | %<Name>
  bus155 : powerlib/Measurements/Load Flow Bus  LConnTagsString=a  ID=bus155  Vbase=150000  Vref=1  Vangle=0  VLF=1  angleLF=0
      settings: AttributesFormatString=|
      | %<ID>
      | %<Vbase>V
      | %<VLF>pu
      | %<angleLF>deg.
      | %<Name>
  bus156 : powerlib/Measurements/Load Flow Bus  LConnTagsString=a  ID=bus156  Vbase=150000  Vref=1  Vangle=0  VLF=1  angleLF=0
      settings: AttributesFormatString=|
      | %<ID>
      | %<Vbase>V
      | %<VLF>pu
      | %<angleLF>deg.
      | %<Name>
  bus157 : powerlib/Measurements/Load Flow Bus  LConnTagsString=a  ID=bus157  Vbase=150000  Vref=1  Vangle=0  VLF=1  angleLF=0
      settings: AttributesFormatString=|
      | %<ID>
      | %<Vbase>V
      | %<VLF>pu
      | %<angleLF>deg.
      | %<Name>
  bus158 : powerlib/Measurements/Load Flow Bus  LConnTagsString=a  ID=bus158  Vbase=150000  Vref=1  Vangle=0  VLF=1  angleLF=0
      settings: AttributesFormatString=|
      | %<ID>
      | %<Vbase>V
      | %<VLF>pu
      | %<angleLF>deg.
      | %<Name>
  bus159 : powerlib/Measurements/Load Flow Bus  LConnTagsString=a  ID=bus159  Vbase=150000  Vref=1  Vangle=0  VLF=1  angleLF=0
      settings: AttributesFormatString=|
      | %<ID>
      | %<Vbase>V
      | %<VLF>pu
      | %<angleLF>deg.
      | %<Name>
  bus16 : powerlib/Measurements/Load Flow Bus  LConnTagsString=a  ID=bus16  Vbase=150000  Vref=1  Vangle=0  VLF=1  angleLF=0
      settings: AttributesFormatString=|
      | %<ID>
      | %<Vbase>V
      | %<VLF>pu
      | %<angleLF>deg.
      | %<Name>
  bus160 : powerlib/Measurements/Load Flow Bus  LConnTagsString=a  ID=bus160  Vbase=220000  Vref=1  Vangle=0  VLF=1  angleLF=0
      settings: AttributesFormatString=|
      | %<ID>
      | %<Vbase>V
      | %<VLF>pu
      | %<angleLF>deg.
      | %<Name>
  bus161 : powerlib/Measurements/Load Flow Bus  LConnTagsString=a  ID=bus161  Vbase=220000  Vref=1  Vangle=0  VLF=1  angleLF=0
      settings: AttributesFormatString=|
      | %<ID>
      | %<Vbase>V
      | %<VLF>pu
      | %<angleLF>deg.
      | %<Name>
  bus162 : powerlib/Measurements/Load Flow Bus  LConnTagsString=a  ID=bus162  Vbase=220000  Vref=1  Vangle=0  VLF=1  angleLF=0
      settings: AttributesFormatString=|
      | %<ID>
      | %<Vbase>V
      | %<VLF>pu
      | %<angleLF>deg.
      | %<Name>
  bus163 : powerlib/Measurements/Load Flow Bus  LConnTagsString=a  ID=bus163  Vbase=220000  Vref=1  Vangle=0  VLF=1  angleLF=0
      settings: AttributesFormatString=|
      | %<ID>
      | %<Vbase>V
      | %<VLF>pu
      | %<angleLF>deg.
      | %<Name>
  bus164 : powerlib/Measurements/Load Flow Bus  LConnTagsString=a  ID=bus164  Vbase=220000  Vref=1  Vangle=0  VLF=1  angleLF=0
      settings: AttributesFormatString=|
      | %<ID>
      | %<Vbase>V
      | %<VLF>pu
      | %<angleLF>deg.
      | %<Name>
  bus165 : powerlib/Measurements/Load Flow Bus  LConnTagsString=a  ID=bus165  Vbase=220000  Vref=1  Vangle=0  VLF=1  angleLF=0
      settings: AttributesFormatString=|
      | %<ID>
      | %<Vbase>V
      | %<VLF>pu
      | %<angleLF>deg.
      | %<Name>
  bus166 : powerlib/Measurements/Load Flow Bus  LConnTagsString=a  ID=bus166  Vbase=220000  Vref=1  Vangle=0  VLF=1  angleLF=0
      settings: AttributesFormatString=|
      | %<ID>
      | %<Vbase>V
      | %<VLF>pu
      | %<angleLF>deg.
      | %<Name>
  bus167 : powerlib/Measurements/Load Flow Bus  LConnTagsString=a  ID=bus167  Vbase=220000  Vref=1  Vangle=0  VLF=1  angleLF=0
      settings: AttributesFormatString=|
      | %<ID>
      | %<Vbase>V
      | %<VLF>pu
      | %<angleLF>deg.
      | %<Name>
  bus168 : powerlib/Measurements/Load Flow Bus  LConnTagsString=a  ID=bus168  Vbase=220000  Vref=1  Vangle=0  VLF=1  angleLF=0
      settings: AttributesFormatString=|
      | %<ID>
      | %<Vbase>V
      | %<VLF>pu
      | %<angleLF>deg.
      | %<Name>
  bus169 : powerlib/Measurements/Load Flow Bus  LConnTagsString=a  ID=bus169  Vbase=220000  Vref=1  Vangle=0  VLF=1  angleLF=0
      settings: AttributesFormatString=|
      | %<ID>
      | %<Vbase>V
      | %<VLF>pu
      | %<angleLF>deg.
      | %<Name>
  bus17 : powerlib/Measurements/Load Flow Bus  LConnTagsString=a  ID=bus17  Vbase=150000  Vref=1  Vangle=0  VLF=1  angleLF=0
      settings: AttributesFormatString=|
      | %<ID>
      | %<Vbase>V
      | %<VLF>pu
      | %<angleLF>deg.
      | %<Name>
  bus170 : powerlib/Measurements/Load Flow Bus  LConnTagsString=a  ID=bus170  Vbase=220000  Vref=1  Vangle=0  VLF=1  angleLF=0
      settings: AttributesFormatString=|
      | %<ID>
      | %<Vbase>V
      | %<VLF>pu
      | %<angleLF>deg.
      | %<Name>
  bus171 : powerlib/Measurements/Load Flow Bus  LConnTagsString=a  ID=bus171  Vbase=220000  Vref=1  Vangle=0  VLF=1  angleLF=0
      settings: AttributesFormatString=|
      | %<ID>
      | %<Vbase>V
      | %<VLF>pu
      | %<angleLF>deg.
      | %<Name>
  bus172 : powerlib/Measurements/Load Flow Bus  LConnTagsString=a  ID=bus172  Vbase=220000  Vref=1  Vangle=0  VLF=1  angleLF=0
      settings: AttributesFormatString=|
      | %<ID>
      | %<Vbase>V
      | %<VLF>pu
      | %<angleLF>deg.
      | %<Name>
  bus173 : powerlib/Measurements/Load Flow Bus  LConnTagsString=a  ID=bus173  Vbase=220000  Vref=1  Vangle=0  VLF=1  angleLF=0
      settings: AttributesFormatString=|
      | %<ID>
      | %<Vbase>V
      | %<VLF>pu
      | %<angleLF>deg.
      | %<Name>
  bus174 : powerlib/Measurements/Load Flow Bus  LConnTagsString=a  ID=bus174  Vbase=220000  Vref=1  Vangle=0  VLF=1  angleLF=0
      settings: AttributesFormatString=|
      | %<ID>
      | %<Vbase>V
      | %<VLF>pu
      | %<angleLF>deg.
      | %<Name>
  bus175 : powerlib/Measurements/Load Flow Bus  LConnTagsString=a  ID=bus175  Vbase=220000  Vref=1  Vangle=0  VLF=1  angleLF=0
      settings: AttributesFormatString=|
      | %<ID>
      | %<Vbase>V
      | %<VLF>pu
      | %<angleLF>deg.
      | %<Name>
  bus176 : powerlib/Measurements/Load Flow Bus  LConnTagsString=a  ID=bus176  Vbase=220000  Vref=1  Vangle=0  VLF=1  angleLF=0
      settings: AttributesFormatString=|
      | %<ID>
      | %<Vbase>V
      | %<VLF>pu
      | %<angleLF>deg.
      | %<Name>
  bus177 : powerlib/Measurements/Load Flow Bus  LConnTagsString=a  ID=bus177  Vbase=220000  Vref=1  Vangle=0  VLF=1  angleLF=0
      settings: AttributesFormatString=|
      | %<ID>
      | %<Vbase>V
      | %<VLF>pu
      | %<angleLF>deg.
      | %<Name>
  bus178 : powerlib/Measurements/Load Flow Bus  LConnTagsString=a  ID=bus178  Vbase=220000  Vref=1  Vangle=0  VLF=1  angleLF=0
      settings: AttributesFormatString=|
      | %<ID>
      | %<Vbase>V
      | %<VLF>pu
      | %<angleLF>deg.
      | %<Name>
  bus179 : powerlib/Measurements/Load Flow Bus  LConnTagsString=a  ID=bus179  Vbase=220000  Vref=1  Vangle=0  VLF=1  angleLF=0
      settings: AttributesFormatString=|
      | %<ID>
      | %<Vbase>V
      | %<VLF>pu
      | %<angleLF>deg.
      | %<Name>
  bus18 : powerlib/Measurements/Load Flow Bus  LConnTagsString=a  ID=bus18  Vbase=150000  Vref=1  Vangle=0  VLF=1  angleLF=0
      settings: AttributesFormatString=|
      | %<ID>
      | %<Vbase>V
      | %<VLF>pu
      | %<angleLF>deg.
      | %<Name>
  bus180 : powerlib/Measurements/Load Flow Bus  LConnTagsString=a  ID=bus180  Vbase=220000  Vref=1  Vangle=0  VLF=1  angleLF=0
      settings: AttributesFormatString=|
      | %<ID>
      | %<Vbase>V
      | %<VLF>pu
      | %<angleLF>deg.
      | %<Name>
  bus181 : powerlib/Measurements/Load Flow Bus  LConnTagsString=a  ID=bus181  Vbase=220000  Vref=1  Vangle=0  VLF=1  angleLF=0
      settings: AttributesFormatString=|
      | %<ID>
      | %<Vbase>V
      | %<VLF>pu
      | %<angleLF>deg.
      | %<Name>
  bus182 : powerlib/Measurements/Load Flow Bus  LConnTagsString=a  ID=bus182  Vbase=220000  Vref=1  Vangle=0  VLF=1  angleLF=0
      settings: AttributesFormatString=|
      | %<ID>
      | %<Vbase>V
      | %<VLF>pu
      | %<angleLF>deg.
      | %<Name>
  bus183 : powerlib/Measurements/Load Flow Bus  LConnTagsString=a  ID=bus183  Vbase=220000  Vref=1  Vangle=0  VLF=1  angleLF=0
      settings: AttributesFormatString=|
      | %<ID>
      | %<Vbase>V
      | %<VLF>pu
      | %<angleLF>deg.
      | %<Name>
  bus184 : powerlib/Measurements/Load Flow Bus  LConnTagsString=a  ID=bus184  Vbase=220000  Vref=1  Vangle=0  VLF=1  angleLF=0
      settings: AttributesFormatString=|
      | %<ID>
      | %<Vbase>V
      | %<VLF>pu
      | %<angleLF>deg.
      | %<Name>
  bus185 : powerlib/Measurements/Load Flow Bus  LConnTagsString=a  ID=bus185  Vbase=220000  Vref=1  Vangle=0  VLF=1  angleLF=0
      settings: AttributesFormatString=|
      | %<ID>
      | %<Vbase>V
      | %<VLF>pu
      | %<angleLF>deg.
      | %<Name>
  bus186 : powerlib/Measurements/Load Flow Bus  LConnTagsString=a  ID=bus186  Vbase=220000  Vref=1  Vangle=0  VLF=1  angleLF=0
      settings: AttributesFormatString=|
      | %<ID>
      | %<Vbase>V
      | %<VLF>pu
      | %<angleLF>deg.
      | %<Name>
  bus187 : powerlib/Measurements/Load Flow Bus  LConnTagsString=a  ID=bus187  Vbase=220000  Vref=1  Vangle=0  VLF=1  angleLF=0
      settings: AttributesFormatString=|
      | %<ID>
      | %<Vbase>V
      | %<VLF>pu
      | %<angleLF>deg.
      | %<Name>
  bus188 : powerlib/Measurements/Load Flow Bus  LConnTagsString=a  ID=bus188  Vbase=220000  Vref=1  Vangle=0  VLF=1  angleLF=0
      settings: AttributesFormatString=|
      | %<ID>
      | %<Vbase>V
      | %<VLF>pu
      | %<angleLF>deg.
      | %<Name>
  bus189 : powerlib/Measurements/Load Flow Bus  LConnTagsString=a  ID=bus189  Vbase=220000  Vref=1  Vangle=0  VLF=1  angleLF=0
      settings: AttributesFormatString=|
      | %<ID>
      | %<Vbase>V
      | %<VLF>pu
      | %<angleLF>deg.
      | %<Name>
  bus19 : powerlib/Measurements/Load Flow Bus  LConnTagsString=a  ID=bus19  Vbase=150000  Vref=1  Vangle=0  VLF=1  angleLF=0
      settings: AttributesFormatString=|
      | %<ID>
      | %<Vbase>V
      | %<VLF>pu
      | %<angleLF>deg.
      | %<Name>
  bus190 : powerlib/Measurements/Load Flow Bus  LConnTagsString=a  ID=bus190  Vbase=220000  Vref=1  Vangle=0  VLF=1  angleLF=0
      settings: AttributesFormatString=|
      | %<ID>
      | %<Vbase>V
      | %<VLF>pu
      | %<angleLF>deg.
      | %<Name>
  bus191 : powerlib/Measurements/Load Flow Bus  LConnTagsString=a  ID=bus191  Vbase=220000  Vref=1  Vangle=0  VLF=1  angleLF=0
      settings: AttributesFormatString=|
      | %<ID>
      | %<Vbase>V
      | %<VLF>pu
      | %<angleLF>deg.
      | %<Name>
  bus192 : powerlib/Measurements/Load Flow Bus  LConnTagsString=a  ID=bus192  Vbase=220000  Vref=1  Vangle=0  VLF=1  angleLF=0
      settings: AttributesFormatString=|
      | %<ID>
      | %<Vbase>V
      | %<VLF>pu
      | %<angleLF>deg.
      | %<Name>
  bus193 : powerlib/Measurements/Load Flow Bus  LConnTagsString=a  ID=bus193  Vbase=220000  Vref=1  Vangle=0  VLF=1  angleLF=0
      settings: AttributesFormatString=|
      | %<ID>
      | %<Vbase>V
      | %<VLF>pu
      | %<angleLF>deg.
      | %<Name>
  bus194 : powerlib/Measurements/Load Flow Bus  LConnTagsString=a  ID=bus194  Vbase=220000  Vref=1  Vangle=0  VLF=1  angleLF=0
      settings: AttributesFormatString=|
      | %<ID>
      | %<Vbase>V
      | %<VLF>pu
      | %<angleLF>deg.
      | %<Name>
  bus195 : powerlib/Measurements/Load Flow Bus  LConnTagsString=a  ID=bus195  Vbase=220000  Vref=1  Vangle=0  VLF=1  angleLF=0
      settings: AttributesFormatString=|
      | %<ID>
      | %<Vbase>V
      | %<VLF>pu
      | %<angleLF>deg.
      | %<Name>
  bus196 : powerlib/Measurements/Load Flow Bus  LConnTagsString=a  ID=bus196  Vbase=220000  Vref=1  Vangle=0  VLF=1  angleLF=0
      settings: AttributesFormatString=|
      | %<ID>
      | %<Vbase>V
      | %<VLF>pu
      | %<angleLF>deg.
      | %<Name>
  bus197 : powerlib/Measurements/Load Flow Bus  LConnTagsString=a  ID=bus197  Vbase=220000  Vref=1  Vangle=0  VLF=1  angleLF=0
      settings: AttributesFormatString=|
      | %<ID>
      | %<Vbase>V
      | %<VLF>pu
      | %<angleLF>deg.
      | %<Name>
  bus198 : powerlib/Measurements/Load Flow Bus  LConnTagsString=a  ID=bus198  Vbase=220000  Vref=1  Vangle=0  VLF=1  angleLF=0
      settings: AttributesFormatString=|
      | %<ID>
      | %<Vbase>V
      | %<VLF>pu
      | %<angleLF>deg.
      | %<Name>
  bus199 : powerlib/Measurements/Load Flow Bus  LConnTagsString=a  ID=bus199  Vbase=220000  Vref=1  Vangle=0  VLF=1  angleLF=0
      settings: AttributesFormatString=|
      | %<ID>
      | %<Vbase>V
      | %<VLF>pu
      | %<angleLF>deg.
      | %<Name>
  bus2 : powerlib/Measurements/Load Flow Bus  LConnTagsString=a  ID=bus2  Vbase=150000  Vref=1  Vangle=0  VLF=1  angleLF=0
      settings: AttributesFormatString=|
      | %<ID>
      | %<Vbase>V
      | %<VLF>pu
      | %<angleLF>deg.
      | %<Name>
  bus20 : powerlib/Measurements/Load Flow Bus  LConnTagsString=a  ID=bus20  Vbase=150000  Vref=1  Vangle=0  VLF=1  angleLF=0
      settings: AttributesFormatString=|
      | %<ID>
      | %<Vbase>V
      | %<VLF>pu
      | %<angleLF>deg.
      | %<Name>
  bus200 : powerlib/Measurements/Load Flow Bus  LConnTagsString=a  ID=bus200  Vbase=220000  Vref=1  Vangle=0  VLF=1  angleLF=0
      settings: AttributesFormatString=|
      | %<ID>
      | %<Vbase>V
      | %<VLF>pu
      | %<angleLF>deg.
      | %<Name>
  bus201 : powerlib/Measurements/Load Flow Bus  LConnTagsString=a  ID=bus201  Vbase=400000  Vref=1  Vangle=0  VLF=1  angleLF=0
      settings: AttributesFormatString=|
      | %<ID>
      | %<Vbase>V
      | %<VLF>pu
      | %<angleLF>deg.
      | %<Name>
  bus202 : powerlib/Measurements/Load Flow Bus  LConnTagsString=a  ID=bus202  Vbase=400000  Vref=1  Vangle=0  VLF=1  angleLF=0
      settings: AttributesFormatString=|
      | %<ID>
      | %<Vbase>V
      | %<VLF>pu
      | %<angleLF>deg.
      | %<Name>
  bus203 : powerlib/Measurements/Load Flow Bus  LConnTagsString=a  ID=bus203  Vbase=400000  Vref=1  Vangle=0  VLF=1  angleLF=0
      settings: AttributesFormatString=|
      | %<ID>
      | %<Vbase>V
      | %<VLF>pu
      | %<angleLF>deg.
      | %<Name>
  bus204 : powerlib/Measurements/Load Flow Bus  LConnTagsString=a  ID=bus204  Vbase=400000  Vref=1  Vangle=0  VLF=1  angleLF=0
      settings: AttributesFormatString=|
      | %<ID>
      | %<Vbase>V
      | %<VLF>pu
      | %<angleLF>deg.
      | %<Name>
  bus205 : powerlib/Measurements/Load Flow Bus  LConnTagsString=a  ID=bus205  Vbase=400000  Vref=1  Vangle=0  VLF=1  angleLF=0
      settings: AttributesFormatString=|
      | %<ID>
      | %<Vbase>V
      | %<VLF>pu
      | %<angleLF>deg.
      | %<Name>
  bus206 : powerlib/Measurements/Load Flow Bus  LConnTagsString=a  ID=bus206  Vbase=400000  Vref=1  Vangle=0  VLF=1  angleLF=0
      settings: AttributesFormatString=|
      | %<ID>
      | %<Vbase>V
      | %<VLF>pu
      | %<angleLF>deg.
      | %<Name>
  bus207 : powerlib/Measurements/Load Flow Bus  LConnTagsString=a  ID=bus207  Vbase=400000  Vref=1  Vangle=0  VLF=1  angleLF=0
      settings: AttributesFormatString=|
      | %<ID>
      | %<Vbase>V
      | %<VLF>pu
      | %<angleLF>deg.
      | %<Name>
  bus208 : powerlib/Measurements/Load Flow Bus  LConnTagsString=a  ID=bus208  Vbase=400000  Vref=1  Vangle=0  VLF=1  angleLF=0
      settings: AttributesFormatString=|
      | %<ID>
      | %<Vbase>V
      | %<VLF>pu
      | %<angleLF>deg.
      | %<Name>
  bus209 : powerlib/Measurements/Load Flow Bus  LConnTagsString=a  ID=bus209  Vbase=400000  Vref=1  Vangle=0  VLF=1  angleLF=0
      settings: AttributesFormatString=|
      | %<ID>
      | %<Vbase>V
      | %<VLF>pu
      | %<angleLF>deg.
      | %<Name>
  bus21 : powerlib/Measurements/Load Flow Bus  LConnTagsString=a  ID=bus21  Vbase=150000  Vref=1  Vangle=0  VLF=1  angleLF=0
      settings: AttributesFormatString=|
      | %<ID>
      | %<Vbase>V
      | %<VLF>pu
      | %<angleLF>deg.
      | %<Name>
  bus210 : powerlib/Measurements/Load Flow Bus  LConnTagsString=a  ID=bus210  Vbase=400000  Vref=1  Vangle=0  VLF=1  angleLF=0
      settings: AttributesFormatString=|
      | %<ID>
      | %<Vbase>V
      | %<VLF>pu
      | %<angleLF>deg.
      | %<Name>
  bus211 : powerlib/Measurements/Load Flow Bus  LConnTagsString=a  ID=bus211  Vbase=400000  Vref=1  Vangle=0  VLF=1  angleLF=0
      settings: AttributesFormatString=|
      | %<ID>
      | %<Vbase>V
      | %<VLF>pu
      | %<angleLF>deg.
      | %<Name>
  bus22 : powerlib/Measurements/Load Flow Bus  LConnTagsString=a  ID=bus22  Vbase=150000  Vref=1  Vangle=0  VLF=1  angleLF=0
      settings: AttributesFormatString=|
      | %<ID>
      | %<Vbase>V
      | %<VLF>pu
      | %<angleLF>deg.
      | %<Name>
  bus23 : powerlib/Measurements/Load Flow Bus  LConnTagsString=a  ID=bus23  Vbase=150000  Vref=1  Vangle=0  VLF=1  angleLF=0
      settings: AttributesFormatString=|
      | %<ID>
      | %<Vbase>V
      | %<VLF>pu
      | %<angleLF>deg.
      | %<Name>
  bus24 : powerlib/Measurements/Load Flow Bus  LConnTagsString=a  ID=bus24  Vbase=150000  Vref=1  Vangle=0  VLF=1  angleLF=0
      settings: AttributesFormatString=|
      | %<ID>
      | %<Vbase>V
      | %<VLF>pu
      | %<angleLF>deg.
      | %<Name>
  bus25 : powerlib/Measurements/Load Flow Bus  LConnTagsString=a  ID=bus25  Vbase=150000  Vref=1  Vangle=0  VLF=1  angleLF=0
      settings: AttributesFormatString=|
      | %<ID>
      | %<Vbase>V
      | %<VLF>pu
      | %<angleLF>deg.
      | %<Name>
  bus26 : powerlib/Measurements/Load Flow Bus  LConnTagsString=a  ID=bus26  Vbase=150000  Vref=1  Vangle=0  VLF=1  angleLF=0
      settings: AttributesFormatString=|
      | %<ID>
      | %<Vbase>V
      | %<VLF>pu
      | %<angleLF>deg.
      | %<Name>
  bus27 : powerlib/Measurements/Load Flow Bus  LConnTagsString=a  ID=bus27  Vbase=150000  Vref=1  Vangle=0  VLF=1  angleLF=0
      settings: AttributesFormatString=|
      | %<ID>
      | %<Vbase>V
      | %<VLF>pu
      | %<angleLF>deg.
      | %<Name>
  bus28 : powerlib/Measurements/Load Flow Bus  LConnTagsString=a  ID=bus28  Vbase=150000  Vref=1  Vangle=0  VLF=1  angleLF=0
      settings: AttributesFormatString=|
      | %<ID>
      | %<Vbase>V
      | %<VLF>pu
      | %<angleLF>deg.
      | %<Name>
  bus29 : powerlib/Measurements/Load Flow Bus  LConnTagsString=a  ID=bus29  Vbase=150000  Vref=1  Vangle=0  VLF=1  angleLF=0
      settings: AttributesFormatString=|
      | %<ID>
      | %<Vbase>V
      | %<VLF>pu
      | %<angleLF>deg.
      | %<Name>
  bus3 : powerlib/Measurements/Load Flow Bus  LConnTagsString=a  ID=bus3  Vbase=150000  Vref=1  Vangle=0  VLF=1  angleLF=0
      settings: AttributesFormatString=|
      | %<ID>
      | %<Vbase>V
      | %<VLF>pu
      | %<angleLF>deg.
      | %<Name>
  bus30 : powerlib/Measurements/Load Flow Bus  LConnTagsString=a  ID=bus30  Vbase=150000  Vref=1  Vangle=0  VLF=1  angleLF=0
      settings: AttributesFormatString=|
      | %<ID>
      | %<Vbase>V
      | %<VLF>pu
      | %<angleLF>deg.
      | %<Name>
  bus31 : powerlib/Measurements/Load Flow Bus  LConnTagsString=a  ID=bus31  Vbase=150000  Vref=1  Vangle=0  VLF=1  angleLF=0
      settings: AttributesFormatString=|
      | %<ID>
      | %<Vbase>V
      | %<VLF>pu
      | %<angleLF>deg.
      | %<Name>
  bus32 : powerlib/Measurements/Load Flow Bus  LConnTagsString=a  ID=bus32  Vbase=150000  Vref=1  Vangle=0  VLF=1  angleLF=0
      settings: AttributesFormatString=|
      | %<ID>
      | %<Vbase>V
      | %<VLF>pu
      | %<angleLF>deg.
      | %<Name>
  bus33 : powerlib/Measurements/Load Flow Bus  LConnTagsString=a  ID=bus33  Vbase=150000  Vref=1  Vangle=0  VLF=1  angleLF=0
      settings: AttributesFormatString=|
      | %<ID>
      | %<Vbase>V
      | %<VLF>pu
      | %<angleLF>deg.
      | %<Name>
  bus34 : powerlib/Measurements/Load Flow Bus  LConnTagsString=a  ID=bus34  Vbase=150000  Vref=1  Vangle=0  VLF=1  angleLF=0
      settings: AttributesFormatString=|
      | %<ID>
      | %<Vbase>V
      | %<VLF>pu
      | %<angleLF>deg.
      | %<Name>
  bus35 : powerlib/Measurements/Load Flow Bus  LConnTagsString=a  ID=bus35  Vbase=150000  Vref=1  Vangle=0  VLF=1  angleLF=0
      settings: AttributesFormatString=|
      | %<ID>
      | %<Vbase>V
      | %<VLF>pu
      | %<angleLF>deg.
      | %<Name>
  bus36 : powerlib/Measurements/Load Flow Bus  LConnTagsString=a  ID=bus36  Vbase=150000  Vref=1  Vangle=0  VLF=1  angleLF=0
      settings: AttributesFormatString=|
      | %<ID>
      | %<Vbase>V
      | %<VLF>pu
      | %<angleLF>deg.
      | %<Name>
  bus37 : powerlib/Measurements/Load Flow Bus  LConnTagsString=a  ID=bus37  Vbase=150000  Vref=1  Vangle=0  VLF=1  angleLF=0
      settings: AttributesFormatString=|
      | %<ID>
      | %<Vbase>V
      | %<VLF>pu
      | %<angleLF>deg.
      | %<Name>
  bus38 : powerlib/Measurements/Load Flow Bus  LConnTagsString=a  ID=bus38  Vbase=150000  Vref=1  Vangle=0  VLF=1  angleLF=0
      settings: AttributesFormatString=|
      | %<ID>
      | %<Vbase>V
      | %<VLF>pu
      | %<angleLF>deg.
      | %<Name>
  bus39 : powerlib/Measurements/Load Flow Bus  LConnTagsString=a  ID=bus39  Vbase=150000  Vref=1  Vangle=0  VLF=1  angleLF=0
      settings: AttributesFormatString=|
      | %<ID>
      | %<Vbase>V
      | %<VLF>pu
      | %<angleLF>deg.
      | %<Name>
  bus4 : powerlib/Measurements/Load Flow Bus  LConnTagsString=a  ID=bus4  Vbase=150000  Vref=1  Vangle=0  VLF=1  angleLF=0
      settings: AttributesFormatString=|
      | %<ID>
      | %<Vbase>V
      | %<VLF>pu
      | %<angleLF>deg.
      | %<Name>
  bus40 : powerlib/Measurements/Load Flow Bus  LConnTagsString=a  ID=bus40  Vbase=150000  Vref=1  Vangle=0  VLF=1  angleLF=0
      settings: AttributesFormatString=|
      | %<ID>
      | %<Vbase>V
      | %<VLF>pu
      | %<angleLF>deg.
      | %<Name>
  bus41 : powerlib/Measurements/Load Flow Bus  LConnTagsString=a  ID=bus41  Vbase=150000  Vref=1  Vangle=0  VLF=1  angleLF=0
      settings: AttributesFormatString=|
      | %<ID>
      | %<Vbase>V
      | %<VLF>pu
      | %<angleLF>deg.
      | %<Name>
  bus42 : powerlib/Measurements/Load Flow Bus  LConnTagsString=a  ID=bus42  Vbase=150000  Vref=1  Vangle=0  VLF=1  angleLF=0
      settings: AttributesFormatString=|
      | %<ID>
      | %<Vbase>V
      | %<VLF>pu
      | %<angleLF>deg.
      | %<Name>
  bus43 : powerlib/Measurements/Load Flow Bus  LConnTagsString=a  ID=bus43  Vbase=150000  Vref=1  Vangle=0  VLF=1  angleLF=0
      settings: AttributesFormatString=|
      | %<ID>
      | %<Vbase>V
      | %<VLF>pu
      | %<angleLF>deg.
      | %<Name>
  bus44 : powerlib/Measurements/Load Flow Bus  LConnTagsString=a  ID=bus44  Vbase=150000  Vref=1  Vangle=0  VLF=1  angleLF=0
      settings: AttributesFormatString=|
      | %<ID>
      | %<Vbase>V
      | %<VLF>pu
      | %<angleLF>deg.
      | %<Name>
  bus45 : powerlib/Measurements/Load Flow Bus  LConnTagsString=a  ID=bus45  Vbase=220000  Vref=1  Vangle=0  VLF=1  angleLF=0
      settings: AttributesFormatString=|
      | %<ID>
      | %<Vbase>V
      | %<VLF>pu
      | %<angleLF>deg.
      | %<Name>
  bus46 : powerlib/Measurements/Load Flow Bus  LConnTagsString=a  ID=bus46  Vbase=220000  Vref=1  Vangle=0  VLF=1  angleLF=0
      settings: AttributesFormatString=|
      | %<ID>
      | %<Vbase>V
      | %<VLF>pu
      | %<angleLF>deg.
      | %<Name>
  bus47 : powerlib/Measurements/Load Flow Bus  LConnTagsString=a  ID=bus47  Vbase=220000  Vref=1  Vangle=0  VLF=1  angleLF=0
      settings: AttributesFormatString=|
      | %<ID>
      | %<Vbase>V
      | %<VLF>pu
      | %<angleLF>deg.
      | %<Name>
  bus48 : powerlib/Measurements/Load Flow Bus  LConnTagsString=a  ID=bus48  Vbase=220000  Vref=1  Vangle=0  VLF=1  angleLF=0
      settings: AttributesFormatString=|
      | %<ID>
      | %<Vbase>V
      | %<VLF>pu
      | %<angleLF>deg.
      | %<Name>
  bus49 : powerlib/Measurements/Load Flow Bus  LConnTagsString=a  ID=bus49  Vbase=220000  Vref=1  Vangle=0  VLF=1  angleLF=0
      settings: AttributesFormatString=|
      | %<ID>
      | %<Vbase>V
      | %<VLF>pu
      | %<angleLF>deg.
      | %<Name>
  bus5 : powerlib/Measurements/Load Flow Bus  LConnTagsString=a  ID=bus5  Vbase=150000  Vref=1  Vangle=0  VLF=1  angleLF=0
      settings: AttributesFormatString=|
      | %<ID>
      | %<Vbase>V
      | %<VLF>pu
      | %<angleLF>deg.
      | %<Name>
  bus50 : powerlib/Measurements/Load Flow Bus  LConnTagsString=a  ID=bus50  Vbase=220000  Vref=1  Vangle=0  VLF=1  angleLF=0
      settings: AttributesFormatString=|
      | %<ID>
      | %<Vbase>V
      | %<VLF>pu
      | %<angleLF>deg.
      | %<Name>
  bus51 : powerlib/Measurements/Load Flow Bus  LConnTagsString=a  ID=bus51  Vbase=220000  Vref=1  Vangle=0  VLF=1  angleLF=0
      settings: AttributesFormatString=|
      | %<ID>
      | %<Vbase>V
      | %<VLF>pu
      | %<angleLF>deg.
      | %<Name>
  bus52 : powerlib/Measurements/Load Flow Bus  LConnTagsString=a  ID=bus52  Vbase=220000  Vref=1  Vangle=0  VLF=1  angleLF=0
      settings: AttributesFormatString=|
      | %<ID>
      | %<Vbase>V
      | %<VLF>pu
      | %<angleLF>deg.
      | %<Name>
  bus53 : powerlib/Measurements/Load Flow Bus  LConnTagsString=a  ID=bus53  Vbase=220000  Vref=1  Vangle=0  VLF=1  angleLF=0
      settings: AttributesFormatString=|
      | %<ID>
      | %<Vbase>V
      | %<VLF>pu
      | %<angleLF>deg.
      | %<Name>
  bus54 : powerlib/Measurements/Load Flow Bus  LConnTagsString=a  ID=bus54  Vbase=220000  Vref=1  Vangle=0  VLF=1  angleLF=0
      settings: AttributesFormatString=|
      | %<ID>
      | %<Vbase>V
      | %<VLF>pu
      | %<angleLF>deg.
      | %<Name>
  bus55 : powerlib/Measurements/Load Flow Bus  LConnTagsString=a  ID=bus55  Vbase=220000  Vref=1  Vangle=0  VLF=1  angleLF=0
      settings: AttributesFormatString=|
      | %<ID>
      | %<Vbase>V
      | %<VLF>pu
      | %<angleLF>deg.
      | %<Name>
  bus56 : powerlib/Measurements/Load Flow Bus  LConnTagsString=a  ID=bus56  Vbase=220000  Vref=1  Vangle=0  VLF=1  angleLF=0
      settings: AttributesFormatString=|
      | %<ID>
      | %<Vbase>V
      | %<VLF>pu
      | %<angleLF>deg.
      | %<Name>
  bus57 : powerlib/Measurements/Load Flow Bus  LConnTagsString=a  ID=bus57  Vbase=220000  Vref=1  Vangle=0  VLF=1  angleLF=0
      settings: AttributesFormatString=|
      | %<ID>
      | %<Vbase>V
      | %<VLF>pu
      | %<angleLF>deg.
      | %<Name>
  bus58 : powerlib/Measurements/Load Flow Bus  LConnTagsString=a  ID=bus58  Vbase=220000  Vref=1  Vangle=0  VLF=1  angleLF=0
      settings: AttributesFormatString=|
      | %<ID>
      | %<Vbase>V
      | %<VLF>pu
      | %<angleLF>deg.
      | %<Name>
  bus59 : powerlib/Measurements/Load Flow Bus  LConnTagsString=a  ID=bus59  Vbase=220000  Vref=1  Vangle=0  VLF=1  angleLF=0
      settings: AttributesFormatString=|
      | %<ID>
      | %<Vbase>V
      | %<VLF>pu
      | %<angleLF>deg.
      | %<Name>
  bus6 : powerlib/Measurements/Load Flow Bus  LConnTagsString=a  ID=bus6  Vbase=150000  Vref=1  Vangle=0  VLF=1  angleLF=0
      settings: AttributesFormatString=|
      | %<ID>
      | %<Vbase>V
      | %<VLF>pu
      | %<angleLF>deg.
      | %<Name>
  bus60 : powerlib/Measurements/Load Flow Bus  LConnTagsString=a  ID=bus60  Vbase=220000  Vref=1  Vangle=0  VLF=1  angleLF=0
      settings: AttributesFormatString=|
      | %<ID>
      | %<Vbase>V
      | %<VLF>pu
      | %<angleLF>deg.
      | %<Name>
  bus61 : powerlib/Measurements/Load Flow Bus  LConnTagsString=a  ID=bus61  Vbase=220000  Vref=1  Vangle=0  VLF=1  angleLF=0
      settings: AttributesFormatString=|
      | %<ID>
      | %<Vbase>V
      | %<VLF>pu
      | %<angleLF>deg.
      | %<Name>
  bus62 : powerlib/Measurements/Load Flow Bus  LConnTagsString=a  ID=bus62  Vbase=220000  Vref=1  Vangle=0  VLF=1  angleLF=0
      settings: AttributesFormatString=|
      | %<ID>
      | %<Vbase>V
      | %<VLF>pu
      | %<angleLF>deg.
      | %<Name>
  bus63 : powerlib/Measurements/Load Flow Bus  LConnTagsString=a  ID=bus63  Vbase=220000  Vref=1  Vangle=0  VLF=1  angleLF=0
      settings: AttributesFormatString=|
      | %<ID>
      | %<Vbase>V
      | %<VLF>pu
      | %<angleLF>deg.
      | %<Name>
  bus64 : powerlib/Measurements/Load Flow Bus  LConnTagsString=a  ID=bus64  Vbase=220000  Vref=1  Vangle=0  VLF=1  angleLF=0
      settings: AttributesFormatString=|
      | %<ID>
      | %<Vbase>V
      | %<VLF>pu
      | %<angleLF>deg.
      | %<Name>
  bus65 : powerlib/Measurements/Load Flow Bus  LConnTagsString=a  ID=bus65  Vbase=220000  Vref=1  Vangle=0  VLF=1  angleLF=0
      settings: AttributesFormatString=|
      | %<ID>
      | %<Vbase>V
      | %<VLF>pu
      | %<angleLF>deg.
      | %<Name>
  bus66 : powerlib/Measurements/Load Flow Bus  LConnTagsString=a  ID=bus66  Vbase=220000  Vref=1  Vangle=0  VLF=1  angleLF=0
      settings: AttributesFormatString=|
      | %<ID>
      | %<Vbase>V
      | %<VLF>pu
      | %<angleLF>deg.
      | %<Name>
  bus67 : powerlib/Measurements/Load Flow Bus  LConnTagsString=a  ID=bus67  Vbase=220000  Vref=1  Vangle=0  VLF=1  angleLF=0
      settings: AttributesFormatString=|
      | %<ID>
      | %<Vbase>V
      | %<VLF>pu
      | %<angleLF>deg.
      | %<Name>
  bus68 : powerlib/Measurements/Load Flow Bus  LConnTagsString=a  ID=bus68  Vbase=220000  Vref=1  Vangle=0  VLF=1  angleLF=0
      settings: AttributesFormatString=|
      | %<ID>
      | %<Vbase>V
      | %<VLF>pu
      | %<angleLF>deg.
      | %<Name>
  bus69 : powerlib/Measurements/Load Flow Bus  LConnTagsString=a  ID=bus69  Vbase=220000  Vref=1  Vangle=0  VLF=1  angleLF=0
      settings: AttributesFormatString=|
      | %<ID>
      | %<Vbase>V
      | %<VLF>pu
      | %<angleLF>deg.
      | %<Name>
  bus7 : powerlib/Measurements/Load Flow Bus  LConnTagsString=a  ID=bus7  Vbase=150000  Vref=1  Vangle=0  VLF=1  angleLF=0
      settings: AttributesFormatString=|
      | %<ID>
      | %<Vbase>V
      | %<VLF>pu
      | %<angleLF>deg.
      | %<Name>
  bus70 : powerlib/Measurements/Load Flow Bus  LConnTagsString=a  ID=bus70  Vbase=220000  Vref=1  Vangle=0  VLF=1  angleLF=0
      settings: AttributesFormatString=|
      | %<ID>
      | %<Vbase>V
      | %<VLF>pu
      | %<angleLF>deg.
      | %<Name>
  bus71 : powerlib/Measurements/Load Flow Bus  LConnTagsString=a  ID=bus71  Vbase=220000  Vref=1  Vangle=0  VLF=1  angleLF=0
      settings: AttributesFormatString=|
      | %<ID>
      | %<Vbase>V
      | %<VLF>pu
      | %<angleLF>deg.
      | %<Name>
  bus72 : powerlib/Measurements/Load Flow Bus  LConnTagsString=a  ID=bus72  Vbase=220000  Vref=1  Vangle=0  VLF=1  angleLF=0
      settings: AttributesFormatString=|
      | %<ID>
      | %<Vbase>V
      | %<VLF>pu
      | %<angleLF>deg.
      | %<Name>
  bus73 : powerlib/Measurements/Load Flow Bus  LConnTagsString=a  ID=bus73  Vbase=220000  Vref=1  Vangle=0  VLF=1  angleLF=0
      settings: AttributesFormatString=|
      | %<ID>
      | %<Vbase>V
      | %<VLF>pu
      | %<angleLF>deg.
      | %<Name>
  bus74 : powerlib/Measurements/Load Flow Bus  LConnTagsString=a  ID=bus74  Vbase=220000  Vref=1  Vangle=0  VLF=1  angleLF=0
      settings: AttributesFormatString=|
      | %<ID>
      | %<Vbase>V
      | %<VLF>pu
      | %<angleLF>deg.
      | %<Name>
  bus75 : powerlib/Measurements/Load Flow Bus  LConnTagsString=a  ID=bus75  Vbase=220000  Vref=1  Vangle=0  VLF=1  angleLF=0
      settings: AttributesFormatString=|
      | %<ID>
      | %<Vbase>V
      | %<VLF>pu
      | %<angleLF>deg.
      | %<Name>
  bus76 : powerlib/Measurements/Load Flow Bus  LConnTagsString=a  ID=bus76  Vbase=220000  Vref=1  Vangle=0  VLF=1  angleLF=0
      settings: AttributesFormatString=|
      | %<ID>
      | %<Vbase>V
      | %<VLF>pu
      | %<angleLF>deg.
      | %<Name>
  bus77 : powerlib/Measurements/Load Flow Bus  LConnTagsString=a  ID=bus77  Vbase=220000  Vref=1  Vangle=0  VLF=1  angleLF=0
      settings: AttributesFormatString=|
      | %<ID>
      | %<Vbase>V
      | %<VLF>pu
      | %<angleLF>deg.
      | %<Name>
  bus78 : powerlib/Measurements/Load Flow Bus  LConnTagsString=a  ID=bus78  Vbase=220000  Vref=1  Vangle=0  VLF=1  angleLF=0
      settings: AttributesFormatString=|
      | %<ID>
      | %<Vbase>V
      | %<VLF>pu
      | %<angleLF>deg.
      | %<Name>
  bus79 : powerlib/Measurements/Load Flow Bus  LConnTagsString=a  ID=bus79  Vbase=220000  Vref=1  Vangle=0  VLF=1  angleLF=0
      settings: AttributesFormatString=|
      | %<ID>
      | %<Vbase>V
      | %<VLF>pu
      | %<angleLF>deg.
      | %<Name>
  bus8 : powerlib/Measurements/Load Flow Bus  LConnTagsString=a  ID=bus8  Vbase=150000  Vref=1  Vangle=0  VLF=1  angleLF=0
      settings: AttributesFormatString=|
      | %<ID>
      | %<Vbase>V
      | %<VLF>pu
      | %<angleLF>deg.
      | %<Name>
  bus80 : powerlib/Measurements/Load Flow Bus  LConnTagsString=a  ID=bus80  Vbase=220000  Vref=1  Vangle=0  VLF=1  angleLF=0
      settings: AttributesFormatString=|
      | %<ID>
      | %<Vbase>V
      | %<VLF>pu
      | %<angleLF>deg.
      | %<Name>
  bus81 : powerlib/Measurements/Load Flow Bus  LConnTagsString=a  ID=bus81  Vbase=220000  Vref=1  Vangle=0  VLF=1  angleLF=0
      settings: AttributesFormatString=|
      | %<ID>
      | %<Vbase>V
      | %<VLF>pu
      | %<angleLF>deg.
      | %<Name>
  bus82 : powerlib/Measurements/Load Flow Bus  LConnTagsString=a  ID=bus82  Vbase=220000  Vref=1  Vangle=0  VLF=1  angleLF=0
      settings: AttributesFormatString=|
      | %<ID>
      | %<Vbase>V
      | %<VLF>pu
      | %<angleLF>deg.
      | %<Name>
  bus83 : powerlib/Measurements/Load Flow Bus  LConnTagsString=a  ID=bus83  Vbase=220000  Vref=1  Vangle=0  VLF=1  angleLF=0
      settings: AttributesFormatString=|
      | %<ID>
      | %<Vbase>V
      | %<VLF>pu
      | %<angleLF>deg.
      | %<Name>
  bus84 : powerlib/Measurements/Load Flow Bus  LConnTagsString=a  ID=bus84  Vbase=220000  Vref=1  Vangle=0  VLF=1  angleLF=0
      settings: AttributesFormatString=|
      | %<ID>
      | %<Vbase>V
      | %<VLF>pu
      | %<angleLF>deg.
      | %<Name>
  bus85 : powerlib/Measurements/Load Flow Bus  LConnTagsString=a  ID=bus85  Vbase=220000  Vref=1  Vangle=0  VLF=1  angleLF=0
      settings: AttributesFormatString=|
      | %<ID>
      | %<Vbase>V
      | %<VLF>pu
      | %<angleLF>deg.
      | %<Name>
  bus86 : powerlib/Measurements/Load Flow Bus  LConnTagsString=a  ID=bus86  Vbase=220000  Vref=1  Vangle=0  VLF=1  angleLF=0
      settings: AttributesFormatString=|
      | %<ID>
      | %<Vbase>V
      | %<VLF>pu
      | %<angleLF>deg.
      | %<Name>
  bus87 : powerlib/Measurements/Load Flow Bus  LConnTagsString=a  ID=bus87  Vbase=220000  Vref=1  Vangle=0  VLF=1  angleLF=0
      settings: AttributesFormatString=|
      | %<ID>
      | %<Vbase>V
      | %<VLF>pu
      | %<angleLF>deg.
      | %<Name>
  bus88 : powerlib/Measurements/Load Flow Bus  LConnTagsString=a  ID=bus88  Vbase=220000  Vref=1  Vangle=0  VLF=1  angleLF=0
      settings: AttributesFormatString=|
      | %<ID>
      | %<Vbase>V
      | %<VLF>pu
      | %<angleLF>deg.
      | %<Name>
  bus89 : powerlib/Measurements/Load Flow Bus  LConnTagsString=a  ID=bus89  Vbase=220000  Vref=1  Vangle=0  VLF=1  angleLF=0
      settings: AttributesFormatString=|
      | %<ID>
      | %<Vbase>V
      | %<VLF>pu
      | %<angleLF>deg.
      | %<Name>
  bus9 : powerlib/Measurements/Load Flow Bus  LConnTagsString=a  ID=bus9  Vbase=150000  Vref=1  Vangle=0  VLF=1  angleLF=0
      settings: AttributesFormatString=|
      | %<ID>
      | %<Vbase>V
      | %<VLF>pu
      | %<angleLF>deg.
      | %<Name>
  bus90 : powerlib/Measurements/Load Flow Bus  LConnTagsString=a  ID=bus90  Vbase=220000  Vref=1  Vangle=0  VLF=1  angleLF=0
      settings: AttributesFormatString=|
      | %<ID>
      | %<Vbase>V
      | %<VLF>pu
      | %<angleLF>deg.
      | %<Name>
  bus91 : powerlib/Measurements/Load Flow Bus  LConnTagsString=a  ID=bus91  Vbase=220000  Vref=1  Vangle=0  VLF=1  angleLF=0
      settings: AttributesFormatString=|
      | %<ID>
      | %<Vbase>V
      | %<VLF>pu
      | %<angleLF>deg.
      | %<Name>
  bus92 : powerlib/Measurements/Load Flow Bus  LConnTagsString=a  ID=bus92  Vbase=220000  Vref=1  Vangle=0  VLF=1  angleLF=0
      settings: AttributesFormatString=|
      | %<ID>
      | %<Vbase>V
      | %<VLF>pu
      | %<angleLF>deg.
      | %<Name>
  bus93 : powerlib/Measurements/Load Flow Bus  LConnTagsString=a  ID=bus93  Vbase=220000  Vref=1  Vangle=0  VLF=1  angleLF=0
      settings: AttributesFormatString=|
      | %<ID>
      | %<Vbase>V
      | %<VLF>pu
      | %<angleLF>deg.
      | %<Name>
  bus94 : powerlib/Measurements/Load Flow Bus  LConnTagsString=a  ID=bus94  Vbase=220000  Vref=1  Vangle=0  VLF=1  angleLF=0
      settings: AttributesFormatString=|
      | %<ID>
      | %<Vbase>V
      | %<VLF>pu
      | %<angleLF>deg.
      | %<Name>
  bus95 : powerlib/Measurements/Load Flow Bus  LConnTagsString=a  ID=bus95  Vbase=220000  Vref=1  Vangle=0  VLF=1  angleLF=0
      settings: AttributesFormatString=|
      | %<ID>
      | %<Vbase>V
      | %<VLF>pu
      | %<angleLF>deg.
      | %<Name>
  bus96 : powerlib/Measurements/Load Flow Bus  LConnTagsString=a  ID=bus96  Vbase=220000  Vref=1  Vangle=0  VLF=1  angleLF=0
      settings: AttributesFormatString=|
      | %<ID>
      | %<Vbase>V
      | %<VLF>pu
      | %<angleLF>deg.
      | %<Name>
  bus97 : powerlib/Measurements/Load Flow Bus  LConnTagsString=a  ID=bus97  Vbase=220000  Vref=1  Vangle=0  VLF=1  angleLF=0
      settings: AttributesFormatString=|
      | %<ID>
      | %<Vbase>V
      | %<VLF>pu
      | %<angleLF>deg.
      | %<Name>
  bus98 : powerlib/Measurements/Load Flow Bus  LConnTagsString=a  ID=bus98  Vbase=220000  Vref=1  Vangle=0  VLF=1  angleLF=0
      settings: AttributesFormatString=|
      | %<ID>
      | %<Vbase>V
      | %<VLF>pu
      | %<angleLF>deg.
      | %<Name>
  bus99 : powerlib/Measurements/Load Flow Bus  LConnTagsString=a  ID=bus99  Vbase=400000  Vref=1  Vangle=0  VLF=1  angleLF=0
      settings: AttributesFormatString=|
      | %<ID>
      | %<Vbase>V
      | %<VLF>pu
      | %<angleLF>deg.
      | %<Name>
  powergui : powerlib/powergui  Priority=1  SimulationMode=Continuous  SolverType=Tustin  SampleTime=50e-6  frequency=60  SPID=off  DisableSnubberDevices=off  DisableRonSwitches=off  DisableVfSwitches=off  SwTol=0  Interpol=off  DisplayEquations=off  Ts=0  methode=off  frequencyindice=60  Pbase=100e6  ErrMax=1e-4  Iterations=50  UnitsV=kV  UnitsW=MW  FunctionMessages=off  echomessages=off  HookPort=off  EnableUseOfTLC=off  x0status=blocks  RestoreLinks=warning  ResistiveCurrentMeasurement=off  Frange=[0:2:500]  Ylog=off  Xlog=on  ShowGrid=off  save=off  variable=ZData  structure=0  ZoomFFT=off  StartTime=0.0  cycles=1  DisplayStyle=1  fundamental=60  FreqAxis=off  MaxFrequency=1000  frequencyindicesteady=1  RmsSteady=1  display=off
  connections:
  T_163204230_150000_Subestação_de_Neves_Corvo/LConn1 -- _CN_163204230_150000_CN_115732510_150000/LConn1
  T_163204230_150000_Subestação_de_Neves_Corvo/LConn2 -- _CN_163204230_150000_CN_115732510_150000/LConn2
  _CN_163204230_150000_CN_115732510_150000/LConn3 -- T_163204230_150000_Subestação_de_Neves_Corvo/LConn3 -- bus1/LConn1
  _CN_163204230_150000_CN_115732510_150000/RConn1 -- T_115732510_150000_Subestação_de_Ourique/LConn1 -- _CN_144622215_150000_CN_115732510_150000/LConn1 -- Linha_150kv_Ourique_Estoi_CN_93512590_150000_CN_115732510_150000/LConn1 -- _CN_163194137_150000_CN_115732510_150000/LConn1 -- _CN_115732510_150000_CN_144635505_150000/LConn1
  _CN_163204230_150000_CN_115732510_150000/RConn2 -- T_115732510_150000_Subestação_de_Ourique/LConn2 -- _CN_144622215_150000_CN_115732510_150000/LConn2 -- Linha_150kv_Ourique_Estoi_CN_93512590_150000_CN_115732510_150000/LConn2 -- _CN_163194137_150000_CN_115732510_150000/LConn2 -- _CN_115732510_150000_CN_144635505_150000/LConn2
  _CN_163204230_150000_CN_115732510_150000/RConn3 -- T_115732510_150000_Subestação_de_Ourique/LConn3 -- _CN_144622215_150000_CN_115732510_150000/LConn3 -- Linha_150kv_Ourique_Estoi_CN_93512590_150000_CN_115732510_150000/LConn3 -- _CN_163194137_150000_CN_115732510_150000/LConn3 -- _CN_115732510_150000_CN_144635505_150000/LConn3 -- bus2/LConn1
  _CN_144622215_150000_CN_109866595_150000/LConn1 -- T_144622215_400000;150000_Subestação_de_Sines/RConn1 -- _CN_144622215_150000_CN_144635505_150000/LConn1 -- _CN_144622215_150000_CN_144635502_150000/LConn1 -- _CN_144622215_150000_CN_163214310_150000/LConn1 -- _CN_144622215_150000_CN_129055610_150000/LConn1 -- _CN_144622215_150000_CN_163214308_150000/LConn1 -- L_144622215/LConn1 -- _CN_144622215_150000_CN_163214309_150000/LConn1 -- _CN_144622215_150000_CN_115732510_150000/RConn1 -- Linha_150kV_Portimão_Saboia_Sines_CN_144622215_150000_CN_163194137_150000/LConn1
  _CN_144622215_150000_CN_109866595_150000/LConn2 -- T_144622215_400000;150000_Subestação_de_Sines/RConn2 -- _CN_144622215_150000_CN_144635505_150000/LConn2 -- _CN_144622215_150000_CN_144635502_150000/LConn2 -- _CN_144622215_150000_CN_163214310_150000/LConn2 -- _CN_144622215_150000_CN_129055610_150000/LConn2 -- _CN_144622215_150000_CN_163214308_150000/LConn2 -- L_144622215/LConn2 -- _CN_144622215_150000_CN_163214309_150000/LConn2 -- _CN_144622215_150000_CN_115732510_150000/RConn2 -- Linha_150kV_Portimão_Saboia_Sines_CN_144622215_150000_CN_163194137_150000/LConn2
  _CN_144622215_150000_CN_109866595_150000/LConn3 -- T_144622215_400000;150000_Subestação_de_Sines/RConn3 -- _CN_144622215_150000_CN_144635505_150000/LConn3 -- _CN_144622215_150000_CN_144635502_150000/LConn3 -- _CN_144622215_150000_CN_163214310_150000/LConn3 -- _CN_144622215_150000_CN_129055610_150000/LConn3 -- _CN_144622215_150000_CN_163214308_150000/LConn3 -- L_144622215/LConn3 -- bus3/LConn1 -- _CN_144622215_150000_CN_163214309_150000/LConn3 -- _CN_144622215_150000_CN_115732510_150000/RConn3 -- Linha_150kV_Portimão_Saboia_Sines_CN_144622215_150000_CN_163194137_150000/LConn3
  _CN_144622215_150000_CN_109866595_150000/RConn1 -- G_109866595_Central_Termoeléctrica_de_Sines/RConn1 -- _CN_144622215_400000_CN_109866595_150000/LConn1
  _CN_144622215_150000_CN_109866595_150000/RConn2 -- G_109866595_Central_Termoeléctrica_de_Sines/RConn2 -- _CN_144622215_400000_CN_109866595_150000/LConn2
  _CN_144622215_150000_CN_109866595_150000/RConn3 -- G_109866595_Central_Termoeléctrica_de_Sines/RConn3 -- _CN_144622215_400000_CN_109866595_150000/LConn3 -- bus4/LConn1
  Linha_150kV_Portimão_Saboia_Sines_CN_144622215_150000_CN_163194137_150000/RConn1 -- T_163194137_400000;150000_Subestação_de_Porto_de_Lagos/LConn1 -- Linha_150kV_Estoi_Porto_de_Lagos_CN_163194137_150000_CN_144711815_150000/LConn1 -- _CN_163194137_150000_CN_115732510_150000/RConn1
  Linha_150kV_Portimão_Saboia_Sines_CN_144622215_150000_CN_163194137_150000/RConn2 -- T_163194137_400000;150000_Subestação_de_Porto_de_Lagos/LConn2 -- Linha_150kV_Estoi_Porto_de_Lagos_CN_163194137_150000_CN_144711815_150000/LConn2 -- _CN_163194137_150000_CN_115732510_150000/RConn2
  Linha_150kV_Portimão_Saboia_Sines_CN_144622215_150000_CN_163194137_150000/RConn3 -- T_163194137_400000;150000_Subestação_de_Porto_de_Lagos/LConn3 -- Linha_150kV_Estoi_Porto_de_Lagos_CN_163194137_150000_CN_144711815_150000/LConn3 -- _CN_163194137_150000_CN_115732510_150000/RConn3 -- bus5/LConn1
  T_163214309__/LConn1 -- _CN_144622215_150000_CN_163214309_150000/RConn1
  T_163214309__/LConn2 -- _CN_144622215_150000_CN_163214309_150000/RConn2
  _CN_144622215_150000_CN_163214309_150000/RConn3 -- T_163214309__/LConn3 -- bus6/LConn1
  _CN_144622215_150000_CN_144635505_150000/RConn1 -- T_144635505_400000;150000_Subestação_de_Ferreira_do_Alentejo/RConn1 -- _CN_115732510_150000_CN_144635505_150000/RConn1 -- _CN_162512815_150000_CN_144635505_150000/LConn1 -- L_144635505/LConn1
  _CN_144622215_150000_CN_144635505_150000/RConn2 -- T_144635505_400000;150000_Subestação_de_Ferreira_do_Alentejo/RConn2 -- _CN_115732510_150000_CN_144635505_150000/RConn2 -- _CN_162512815_150000_CN_144635505_150000/LConn2 -- L_144635505/LConn2
  _CN_144622215_150000_CN_144635505_150000/RConn3 -- T_144635505_400000;150000_Subestação_de_Ferreira_do_Alentejo/RConn3 -- _CN_115732510_150000_CN_144635505_150000/RConn3 -- _CN_162512815_150000_CN_144635505_150000/LConn3 -- L_144635505/LConn3 -- bus7/LConn1
  T_144635502_150000_Subestação_de_Ermidas_Sado/LConn1 -- _CN_144622215_150000_CN_144635502_150000/RConn1
  T_144635502_150000_Subestação_de_Ermidas_Sado/LConn2 -- _CN_144622215_150000_CN_144635502_150000/RConn2
  _CN_144622215_150000_CN_144635502_150000/RConn3 -- T_144635502_150000_Subestação_de_Ermidas_Sado/LConn3 -- bus8/LConn1
  T_163214310_150000_/LConn1 -- _CN_144622215_150000_CN_163214310_150000/RConn1
  T_163214310_150000_/LConn2 -- _CN_144622215_150000_CN_163214310_150000/RConn2
  _CN_144622215_150000_CN_163214310_150000/RConn3 -- T_163214310_150000_/LConn3 -- bus9/LConn1
  _CN_144622215_150000_CN_129055610_150000/RConn1 -- T_129055610_400000;150000_Subestação_de_Palmela/RConn1 -- _CN_163226990_150000_CN_129055610_150000/LConn1 -- _CN_171253574_150000_CN_129055610_150000/LConn1 -- _CN_132614219_150000_CN_129055610_150000/LConn1 -- _CN_156176120_150000_CN_129055610_150000/LConn1 -- L_129055610/LConn1
  _CN_144622215_150000_CN_129055610_150000/RConn2 -- T_129055610_400000;150000_Subestação_de_Palmela/RConn2 -- _CN_163226990_150000_CN_129055610_150000/LConn2 -- _CN_171253574_150000_CN_129055610_150000/LConn2 -- _CN_132614219_150000_CN_129055610_150000/LConn2 -- _CN_156176120_150000_CN_129055610_150000/LConn2 -- L_129055610/LConn2
  _CN_144622215_150000_CN_129055610_150000/RConn3 -- T_129055610_400000;150000_Subestação_de_Palmela/RConn3 -- _CN_163226990_150000_CN_129055610_150000/LConn3 -- _CN_171253574_150000_CN_129055610_150000/LConn3 -- _CN_132614219_150000_CN_129055610_150000/LConn3 -- _CN_156176120_150000_CN_129055610_150000/LConn3 -- L_129055610/LConn3 -- bus10/LConn1
  T_163214308__/LConn1 -- _CN_144622215_150000_CN_163214308_150000/RConn1
  T_163214308__/LConn2 -- _CN_144622215_150000_CN_163214308_150000/RConn2
  _CN_144622215_150000_CN_163214308_150000/RConn3 -- T_163214308__/LConn3 -- bus11/LConn1
  _CN_24636044_150000_CN_402947133_150000/LConn1 -- T_24636044_400000;220000;150000_Subestação_de_Fanhões/RConn4 -- L_24636044/LConn1
  _CN_24636044_150000_CN_402947133_150000/LConn2 -- T_24636044_400000;220000;150000_Subestação_de_Fanhões/RConn5 -- L_24636044/LConn2
  _CN_24636044_150000_CN_402947133_150000/LConn3 -- T_24636044_400000;220000;150000_Subestação_de_Fanhões/RConn6 -- L_24636044/LConn3 -- bus12/LConn1
  _CN_24636044_150000_CN_402947133_150000/RConn1 -- T_402947133_220000_Subestação_de_Sacavém/RConn1 -- L_402947133/LConn1
  _CN_24636044_150000_CN_402947133_150000/RConn2 -- T_402947133_220000_Subestação_de_Sacavém/RConn2 -- L_402947133/LConn2
  _CN_24636044_150000_CN_402947133_150000/RConn3 -- T_402947133_220000_Subestação_de_Sacavém/RConn3 -- L_402947133/LConn3 -- bus13/LConn1
  T_163227021_150000;60000_Subestação_de_Trafaria/LConn1 -- _CN_163227021_150000_CN_171253574_150000/LConn1
  T_163227021_150000;60000_Subestação_de_Trafaria/LConn2 -- _CN_163227021_150000_CN_171253574_150000/LConn2
  _CN_163227021_150000_CN_171253574_150000/LConn3 -- T_163227021_150000;60000_Subestação_de_Trafaria/LConn3 -- bus14/LConn1
  _CN_163227021_150000_CN_171253574_150000/RConn1 -- T_171253574_150000_/LConn1 -- _CN_163226990_150000_CN_171253574_150000/LConn1 -- _CN_171253574_150000_CN_163226993_150000/LConn1 -- _CN_171253574_150000_CN_129055610_150000/RConn1
  _CN_163227021_150000_CN_171253574_150000/RConn2 -- T_171253574_150000_/LConn2 -- _CN_163226990_150000_CN_171253574_150000/LConn2 -- _CN_171253574_150000_CN_163226993_150000/LConn2 -- _CN_171253574_150000_CN_129055610_150000/RConn2
  _CN_163227021_150000_CN_171253574_150000/RConn3 -- T_171253574_150000_/LConn3 -- _CN_163226990_150000_CN_171253574_150000/LConn3 -- _CN_171253574_150000_CN_163226993_150000/LConn3 -- _CN_171253574_150000_CN_129055610_150000/RConn3 -- bus15/LConn1
  Linha_150kv_Ourique_Estoi_CN_93512590_150000_CN_201459319_150000/LConn1 -- T_93512590_150000;60000_Subestação_de_Estoi/LConn1 -- Linha_150kv_Ourique_Estoi_CN_93512590_150000_CN_115732510_150000/RConn1 -- Linha_150_KV_Tunes–Estoi_CN_93512590_150000_CN_144711815_150000/LConn1
  Linha_150kv_Ourique_Estoi_CN_93512590_150000_CN_201459319_150000/LConn2 -- T_93512590_150000;60000_Subestação_de_Estoi/LConn2 -- Linha_150kv_Ourique_Estoi_CN_93512590_150000_CN_115732510_150000/RConn2 -- Linha_150_KV_Tunes–Estoi_CN_93512590_150000_CN_144711815_150000/LConn2
  Linha_150kv_Ourique_Estoi_CN_93512590_150000_CN_201459319_150000/LConn3 -- T_93512590_150000;60000_Subestação_de_Estoi/LConn3 -- Linha_150kv_Ourique_Estoi_CN_93512590_150000_CN_115732510_150000/RConn3 -- Linha_150_KV_Tunes–Estoi_CN_93512590_150000_CN_144711815_150000/LConn3 -- bus16/LConn1
  T_201459319_400000;150000_Subestação_REN_Casas_Baixas/LConn1 -- Linha_150kv_Ourique_Estoi_CN_93512590_150000_CN_201459319_150000/RConn1
  T_201459319_400000;150000_Subestação_REN_Casas_Baixas/LConn2 -- Linha_150kv_Ourique_Estoi_CN_93512590_150000_CN_201459319_150000/RConn2
  Linha_150kv_Ourique_Estoi_CN_93512590_150000_CN_201459319_150000/RConn3 -- T_201459319_400000;150000_Subestação_REN_Casas_Baixas/LConn3 -- bus17/LConn1
  Linha_150_KV_Tunes–Estoi_CN_93512590_150000_CN_144711815_150000/RConn1 -- T_144711815_150000;60000_Subestação_de_Tunes/LConn1 -- Linha_150kV_Estoi_Porto_de_Lagos_CN_163194137_150000_CN_144711815_150000/RConn1
  Linha_150_KV_Tunes–Estoi_CN_93512590_150000_CN_144711815_150000/RConn2 -- T_144711815_150000;60000_Subestação_de_Tunes/LConn2 -- Linha_150kV_Estoi_Porto_de_Lagos_CN_163194137_150000_CN_144711815_150000/RConn2
  Linha_150_KV_Tunes–Estoi_CN_93512590_150000_CN_144711815_150000/RConn3 -- T_144711815_150000;60000_Subestação_de_Tunes/LConn3 -- Linha_150kV_Estoi_Porto_de_Lagos_CN_163194137_150000_CN_144711815_150000/RConn3 -- bus18/LConn1
  _CN_151061905_150000_CN_151061928_150000/LConn1 -- T_151061905_150000_Subestação_de_Oleiros/LConn1 -- _CN_151061905_150000_CN_383950755_150000/LConn1 -- _CN_151061905_150000_CN_100898242_150000/LConn1 -- _CN_151061905_150000_CN_132865612_150000/LConn1 -- _CN_151061905_150000_CN_151061884_150000/LConn1
  _CN_151061905_150000_CN_151061928_150000/LConn2 -- T_151061905_150000_Subestação_de_Oleiros/LConn2 -- _CN_151061905_150000_CN_383950755_150000/LConn2 -- _CN_151061905_150000_CN_100898242_150000/LConn2 -- _CN_151061905_150000_CN_132865612_150000/LConn2 -- _CN_151061905_150000_CN_151061884_150000/LConn2
  _CN_151061905_150000_CN_151061928_150000/LConn3 -- T_151061905_150000_Subestação_de_Oleiros/LConn3 -- _CN_151061905_150000_CN_383950755_150000/LConn3 -- _CN_151061905_150000_CN_100898242_150000/LConn3 -- _CN_151061905_150000_CN_132865612_150000/LConn3 -- _CN_151061905_150000_CN_151061884_150000/LConn3 -- bus19/LConn1
  _CN_151061905_150000_CN_151061928_150000/RConn1 -- T_151061928_150000;60000_Subestação_de_Vila_Fria/LConn1 -- _CN_151061928_150000_CN_151077584_150000/LConn1
  _CN_151061905_150000_CN_151061928_150000/RConn2 -- T_151061928_150000;60000_Subestação_de_Vila_Fria/LConn2 -- _CN_151061928_150000_CN_151077584_150000/LConn2
  _CN_151061905_150000_CN_151061928_150000/RConn3 -- T_151061928_150000;60000_Subestação_de_Vila_Fria/LConn3 -- _CN_151061928_150000_CN_151077584_150000/LConn3 -- bus20/LConn1
  _CN_151061905_150000_CN_383950755_150000/RConn1 -- G_383950755_Barragem_da_Venda_Nova/RConn1 -- _CN_151077578_150000_CN_383950755_150000/LConn1
  _CN_151061905_150000_CN_383950755_150000/RConn2 -- G_383950755_Barragem_da_Venda_Nova/RConn2 -- _CN_151077578_150000_CN_383950755_150000/LConn2
  _CN_151061905_150000_CN_383950755_150000/RConn3 -- G_383950755_Barragem_da_Venda_Nova/RConn3 -- _CN_151077578_150000_CN_383950755_150000/LConn3 -- bus21/LConn1
  _CN_151061905_150000_CN_100898242_150000/RConn1 -- T_100898242_150000;60000_Subestação_de_Ermesinde/LConn1 -- _CN_151109816_150000_CN_100898242_150000/LConn1 -- _CN_100898242_150000_CN_142182853_150000/LConn1 -- _CN_100898242_150000_CN_132865612_150000/LConn1
  _CN_151061905_150000_CN_100898242_150000/RConn2 -- T_100898242_150000;60000_Subestação_de_Ermesinde/LConn2 -- _CN_151109816_150000_CN_100898242_150000/LConn2 -- _CN_100898242_150000_CN_142182853_150000/LConn2 -- _CN_100898242_150000_CN_132865612_150000/LConn2
  _CN_151061905_150000_CN_100898242_150000/RConn3 -- T_100898242_150000;60000_Subestação_de_Ermesinde/LConn3 -- _CN_151109816_150000_CN_100898242_150000/LConn3 -- _CN_100898242_150000_CN_142182853_150000/LConn3 -- _CN_100898242_150000_CN_132865612_150000/LConn3 -- bus22/LConn1
  _CN_151061905_150000_CN_132865612_150000/RConn1 -- T_132865612_400000;150000;60000_Subestação_de_Riba_de_Ave/RConn1 -- _CN_132865612_150000_CN_151084399_150000/LConn1 -- _CN_132865612_150000_CN_151077584_150000/LConn1 -- L_132865612/LConn1 -- _CN_151090496_150000_CN_132865612_150000/LConn1 -- _CN_100898242_150000_CN_132865612_150000/RConn1
  _CN_151061905_150000_CN_132865612_150000/RConn2 -- T_132865612_400000;150000;60000_Subestação_de_Riba_de_Ave/RConn2 -- _CN_132865612_150000_CN_151084399_150000/LConn2 -- _CN_132865612_150000_CN_151077584_150000/LConn2 -- L_132865612/LConn2 -- _CN_151090496_150000_CN_132865612_150000/LConn2 -- _CN_100898242_150000_CN_132865612_150000/RConn2
  _CN_151061905_150000_CN_132865612_150000/RConn3 -- T_132865612_400000;150000;60000_Subestação_de_Riba_de_Ave/RConn3 -- _CN_132865612_150000_CN_151084399_150000/LConn3 -- _CN_132865612_150000_CN_151077584_150000/LConn3 -- L_132865612/LConn3 -- bus23/LConn1 -- _CN_151090496_150000_CN_132865612_150000/LConn3 -- _CN_100898242_150000_CN_132865612_150000/RConn3
  _CN_151061905_150000_CN_151061884_150000/RConn1 -- T_151061884_400000;15000_Subestação_de_Pedralva/RConn1 -- _CN_151061920_150000_CN_151061884_150000/LConn1 -- _CN_151077584_150000_CN_151061884_150000/LConn1 -- L_151061884/LConn1
  _CN_151061905_150000_CN_151061884_150000/RConn2 -- T_151061884_400000;15000_Subestação_de_Pedralva/RConn2 -- _CN_151061920_150000_CN_151061884_150000/LConn2 -- _CN_151077584_150000_CN_151061884_150000/LConn2 -- L_151061884/LConn2
  _CN_151061905_150000_CN_151061884_150000/RConn3 -- T_151061884_400000;15000_Subestação_de_Pedralva/RConn3 -- _CN_151061920_150000_CN_151061884_150000/LConn3 -- _CN_151077584_150000_CN_151061884_150000/LConn3 -- L_151061884/LConn3 -- bus24/LConn1
  _CN_163226990_150000_CN_171253574_150000/RConn1 -- T_163226990_150000_/LConn1 -- _CN_163226990_150000_CN_129055610_150000/RConn1
  _CN_163226990_150000_CN_171253574_150000/RConn2 -- T_163226990_150000_/LConn2 -- _CN_163226990_150000_CN_129055610_150000/RConn2
  _CN_163226990_150000_CN_171253574_150000/RConn3 -- T_163226990_150000_/LConn3 -- _CN_163226990_150000_CN_129055610_150000/RConn3 -- bus25/LConn1
  T_151061920_150000_/LConn1 -- _CN_151061920_150000_CN_151061884_150000/RConn1
  T_151061920_150000_/LConn2 -- _CN_151061920_150000_CN_151061884_150000/RConn2
  _CN_151061920_150000_CN_151061884_150000/RConn3 -- T_151061920_150000_/LConn3 -- bus26/LConn1
  T_163226982_150000_Subestação_de_Pegões/LConn1 -- _CN_163226982_150000_CN_162512815_150000/LConn1
  T_163226982_150000_Subestação_de_Pegões/LConn2 -- _CN_163226982_150000_CN_162512815_150000/LConn2
  _CN_163226982_150000_CN_162512815_150000/LConn3 -- T_163226982_150000_Subestação_de_Pegões/LConn3 -- bus27/LConn1
  _CN_163226982_150000_CN_162512815_150000/RConn1 -- T_162512815_150000;60000_Subestação_de_Évora/LConn1 -- _CN_162512815_150000_CN_144635505_150000/RConn1
  _CN_163226982_150000_CN_162512815_150000/RConn2 -- T_162512815_150000;60000_Subestação_de_Évora/LConn2 -- _CN_162512815_150000_CN_144635505_150000/RConn2
  _CN_163226982_150000_CN_162512815_150000/RConn3 -- T_162512815_150000;60000_Subestação_de_Évora/LConn3 -- _CN_162512815_150000_CN_144635505_150000/RConn3 -- bus28/LConn1
  T_151069425_150000_/LConn1 -- _CN_151069425_150000_CN_151077584_150000/LConn1
  T_151069425_150000_/LConn2 -- _CN_151069425_150000_CN_151077584_150000/LConn2
  _CN_151069425_150000_CN_151077584_150000/LConn3 -- T_151069425_150000_/LConn3 -- bus29/LConn1
  _CN_151069425_150000_CN_151077584_150000/RConn1 -- T_151077584_150000_/LConn1 -- _CN_151077584_150000_CN_151061884_150000/RConn1 -- _CN_151077578_150000_CN_151077584_150000/LConn1 -- _CN_132865612_150000_CN_151077584_150000/RConn1 -- _CN_151061928_150000_CN_151077584_150000/RConn1
  _CN_151069425_150000_CN_151077584_150000/RConn2 -- T_151077584_150000_/LConn2 -- _CN_151077584_150000_CN_151061884_150000/RConn2 -- _CN_151077578_150000_CN_151077584_150000/LConn2 -- _CN_132865612_150000_CN_151077584_150000/RConn2 -- _CN_151061928_150000_CN_151077584_150000/RConn2
  _CN_151069425_150000_CN_151077584_150000/RConn3 -- T_151077584_150000_/LConn3 -- _CN_151077584_150000_CN_151061884_150000/RConn3 -- bus30/LConn1 -- _CN_151077578_150000_CN_151077584_150000/LConn3 -- _CN_132865612_150000_CN_151077584_150000/RConn3 -- _CN_151061928_150000_CN_151077584_150000/RConn3
  T_151109816__/LConn1 -- _CN_151109816_150000_CN_100898242_150000/RConn1
  T_151109816__/LConn2 -- _CN_151109816_150000_CN_100898242_150000/RConn2
  _CN_151109816_150000_CN_100898242_150000/RConn3 -- T_151109816__/LConn3 -- bus31/LConn1
  T_151090496_150000;60000_Subestação_de_Ruivães/LConn1 -- _CN_151090496_150000_CN_132865612_150000/RConn1
  T_151090496_150000;60000_Subestação_de_Ruivães/LConn2 -- _CN_151090496_150000_CN_132865612_150000/RConn2
  _CN_151090496_150000_CN_132865612_150000/RConn3 -- T_151090496_150000;60000_Subestação_de_Ruivães/LConn3 -- bus32/LConn1
  T_165898049_150000_/LConn1 -- _CN_165898049_150000_CN_132614219_150000/LConn1
  T_165898049_150000_/LConn2 -- _CN_165898049_150000_CN_132614219_150000/LConn2
  _CN_165898049_150000_CN_132614219_150000/LConn3 -- T_165898049_150000_/LConn3 -- bus33/LConn1
  _CN_165898049_150000_CN_132614219_150000/RConn1 -- T_132614219_150000_/LConn1 -- _CN_144762180_150000_CN_132614219_150000/LConn1 -- _CN_132614219_150000_CN_129055610_150000/RConn1
  _CN_165898049_150000_CN_132614219_150000/RConn2 -- T_132614219_150000_/LConn2 -- _CN_144762180_150000_CN_132614219_150000/LConn2 -- _CN_132614219_150000_CN_129055610_150000/RConn2
  _CN_165898049_150000_CN_132614219_150000/RConn3 -- T_132614219_150000_/LConn3 -- _CN_144762180_150000_CN_132614219_150000/LConn3 -- _CN_132614219_150000_CN_129055610_150000/RConn3 -- bus34/LConn1
  _CN_100898242_150000_CN_142182853_150000/RConn1 -- T_142182853_220000;150000;60000_Subestação_de_Vermoim/RConn1 -- L_142182853/LConn1
  _CN_100898242_150000_CN_142182853_150000/RConn2 -- T_142182853_220000;150000;60000_Subestação_de_Vermoim/RConn2 -- L_142182853/LConn2
  _CN_100898242_150000_CN_142182853_150000/RConn3 -- T_142182853_220000;150000;60000_Subestação_de_Vermoim/RConn3 -- L_142182853/LConn3 -- bus35/LConn1
  _CN_144762180_150000_CN_132614219_150000/RConn1 -- T_144762180_220000_/RConn1 -- L_144762180/LConn1
  _CN_144762180_150000_CN_132614219_150000/RConn2 -- T_144762180_220000_/RConn2 -- L_144762180/LConn2
  _CN_144762180_150000_CN_132614219_150000/RConn3 -- T_144762180_220000_/RConn3 -- L_144762180/LConn3 -- bus36/LConn1
  T_163226993_150000_Fogueteiro/LConn1 -- _CN_171253574_150000_CN_163226993_150000/RConn1
  T_163226993_150000_Fogueteiro/LConn2 -- _CN_171253574_150000_CN_163226993_150000/RConn2
  _CN_171253574_150000_CN_163226993_150000/RConn3 -- T_163226993_150000_Fogueteiro/LConn3 -- bus37/LConn1
  T_151077580_150000_/LConn1 -- _CN_151077580_150000_CN_151077578_150000/LConn1
  T_151077580_150000_/LConn2 -- _CN_151077580_150000_CN_151077578_150000/LConn2
  _CN_151077580_150000_CN_151077578_150000/LConn3 -- T_151077580_150000_/LConn3 -- bus38/LConn1
  _CN_151077580_150000_CN_151077578_150000/RConn1 -- T_151077578_150000;60000_/LConn1 -- _CN_151077578_150000_CN_397005282_150000/LConn1 -- _CN_151077578_150000_CN_383950755_150000/RConn1 -- _CN_151077578_150000_CN_151077584_150000/RConn1
  _CN_151077580_150000_CN_151077578_150000/RConn2 -- T_151077578_150000;60000_/LConn2 -- _CN_151077578_150000_CN_397005282_150000/LConn2 -- _CN_151077578_150000_CN_383950755_150000/RConn2 -- _CN_151077578_150000_CN_151077584_150000/RConn2
  _CN_151077580_150000_CN_151077578_150000/RConn3 -- T_151077578_150000;60000_/LConn3 -- _CN_151077578_150000_CN_397005282_150000/LConn3 -- _CN_151077578_150000_CN_383950755_150000/RConn3 -- _CN_151077578_150000_CN_151077584_150000/RConn3 -- bus39/LConn1
  T_397005282__/LConn1 -- _CN_151077578_150000_CN_397005282_150000/RConn1
  T_397005282__/LConn2 -- _CN_151077578_150000_CN_397005282_150000/RConn2
  _CN_151077578_150000_CN_397005282_150000/RConn3 -- T_397005282__/LConn3 -- bus40/LConn1
  T_151084399_150000_/LConn1 -- _CN_132865612_150000_CN_151084399_150000/RConn1
  T_151084399_150000_/LConn2 -- _CN_132865612_150000_CN_151084399_150000/RConn2
  _CN_132865612_150000_CN_151084399_150000/RConn3 -- T_151084399_150000_/LConn3 -- bus41/LConn1
  T_163195990_150000_Subestação_de_Saboia/LConn1 -- _CN_163195990_150000_CN_163195991_150000/LConn1
  T_163195990_150000_Subestação_de_Saboia/LConn2 -- _CN_163195990_150000_CN_163195991_150000/LConn2
  _CN_163195990_150000_CN_163195991_150000/LConn3 -- T_163195990_150000_Subestação_de_Saboia/LConn3 -- bus42/LConn1
  T_163195991_150000_Subestação_de_Luzianes/LConn1 -- _CN_163195990_150000_CN_163195991_150000/RConn1
  T_163195991_150000_Subestação_de_Luzianes/LConn2 -- _CN_163195990_150000_CN_163195991_150000/RConn2
  _CN_163195990_150000_CN_163195991_150000/RConn3 -- T_163195991_150000_Subestação_de_Luzianes/LConn3 -- bus43/LConn1
  T_156176120_150000;60000_/LConn1 -- _CN_156176120_150000_CN_129055610_150000/RConn1
  T_156176120_150000;60000_/LConn2 -- _CN_156176120_150000_CN_129055610_150000/RConn2
  _CN_156176120_150000_CN_129055610_150000/RConn3 -- T_156176120_150000;60000_/LConn3 -- bus44/LConn1
  _CN_144400130_220000_CN_144374439_220000/LConn1 -- T_144400130_220000_/LConn1 -- _CN_144400130_220000_CN_124722161_220000/LConn1
  _CN_144400130_220000_CN_144374439_220000/LConn2 -- T_144400130_220000_/LConn2 -- _CN_144400130_220000_CN_124722161_220000/LConn2
  _CN_144400130_220000_CN_144374439_220000/LConn3 -- T_144400130_220000_/LConn3 -- _CN_144400130_220000_CN_124722161_220000/LConn3 -- bus45/LConn1
  _CN_144400130_220000_CN_144374439_220000/RConn1 -- T_144374439_220000_/LConn1 -- _CN_144396420_220000_CN_144374439_220000/LConn1 -- _CN_151162379_220000_CN_144374439_220000/LConn1 -- _CN_127205653_220000_CN_144374439_220000/LConn1 -- _CN_144374439_220000_CN_144374442_220000/LConn1
  _CN_144400130_220000_CN_144374439_220000/RConn2 -- T_144374439_220000_/LConn2 -- _CN_144396420_220000_CN_144374439_220000/LConn2 -- _CN_151162379_220000_CN_144374439_220000/LConn2 -- _CN_127205653_220000_CN_144374439_220000/LConn2 -- _CN_144374439_220000_CN_144374442_220000/LConn2
  _CN_144400130_220000_CN_144374439_220000/RConn3 -- T_144374439_220000_/LConn3 -- _CN_144396420_220000_CN_144374439_220000/LConn3 -- _CN_151162379_220000_CN_144374439_220000/LConn3 -- _CN_127205653_220000_CN_144374439_220000/LConn3 -- _CN_144374439_220000_CN_144374442_220000/LConn3 -- bus46/LConn1
  _CN_144400130_220000_CN_124722161_220000/RConn1 -- T_124722161_400000;220000;60000_Subestação_de_Recarei/RConn1 -- _CN_144396420_220000_CN_124722161_220000/LConn1 -- _CN_142658477_220000_CN_124722161_220000/LConn1 -- _CN_142182853_220000_CN_124722161_220000/LConn1 -- L_124722161/LConn1
  _CN_144400130_220000_CN_124722161_220000/RConn2 -- T_124722161_400000;220000;60000_Subestação_de_Recarei/RConn2 -- _CN_144396420_220000_CN_124722161_220000/LConn2 -- _CN_142658477_220000_CN_124722161_220000/LConn2 -- _CN_142182853_220000_CN_124722161_220000/LConn2 -- L_124722161/LConn2
  _CN_144400130_220000_CN_124722161_220000/RConn3 -- T_124722161_400000;220000;60000_Subestação_de_Recarei/RConn3 -- _CN_144396420_220000_CN_124722161_220000/LConn3 -- _CN_142658477_220000_CN_124722161_220000/LConn3 -- _CN_142182853_220000_CN_124722161_220000/LConn3 -- L_124722161/LConn3 -- bus47/LConn1
  _CN_144396420_220000_CN_144398555_220000/LConn1 -- T_144396420_220000;60000_Subestação_de_Régua/LConn1 -- _CN_144396420_220000_CN_144396428_220000/LConn1 -- _CN_144396420_220000_CN_144374439_220000/RConn1 -- _CN_144396420_220000_CN_127205502_220000/LConn1 -- _CN_144396420_220000_CN_144396412_220000/LConn1 -- _CN_144396420_220000_CN_124722161_220000/RConn1 -- _CN_144396420_220000_CN_126366408_220000/LConn1
  _CN_144396420_220000_CN_144398555_220000/LConn2 -- T_144396420_220000;60000_Subestação_de_Régua/LConn2 -- _CN_144396420_220000_CN_144396428_220000/LConn2 -- _CN_144396420_220000_CN_144374439_220000/RConn2 -- _CN_144396420_220000_CN_127205502_220000/LConn2 -- _CN_144396420_220000_CN_144396412_220000/LConn2 -- _CN_144396420_220000_CN_124722161_220000/RConn2 -- _CN_144396420_220000_CN_126366408_220000/LConn2
  _CN_144396420_220000_CN_144398555_220000/LConn3 -- T_144396420_220000;60000_Subestação_de_Régua/LConn3 -- _CN_144396420_220000_CN_144396428_220000/LConn3 -- bus48/LConn1 -- _CN_144396420_220000_CN_144374439_220000/RConn3 -- _CN_144396420_220000_CN_127205502_220000/LConn3 -- _CN_144396420_220000_CN_144396412_220000/LConn3 -- _CN_144396420_220000_CN_124722161_220000/RConn3 -- _CN_144396420_220000_CN_126366408_220000/LConn3
  T_144398555_220000_Subestação_de_Vila_Pouca_de_Aguiar/LConn1 -- _CN_144396420_220000_CN_144398555_220000/RConn1
  T_144398555_220000_Subestação_de_Vila_Pouca_de_Aguiar/LConn2 -- _CN_144396420_220000_CN_144398555_220000/RConn2
  _CN_144396420_220000_CN_144398555_220000/RConn3 -- T_144398555_220000_Subestação_de_Vila_Pouca_de_Aguiar/LConn3 -- bus49/LConn1
  T_126366408_220000;60000_Subestação_de_Urrô/LConn1 -- _CN_144396420_220000_CN_126366408_220000/RConn1
  T_126366408_220000;60000_Subestação_de_Urrô/LConn2 -- _CN_144396420_220000_CN_126366408_220000/RConn2
  _CN_144396420_220000_CN_126366408_220000/RConn3 -- T_126366408_220000;60000_Subestação_de_Urrô/LConn3 -- bus50/LConn1
  _CN_144396420_220000_CN_127205502_220000/RConn1 -- T_127205502_220000_Subestação_de_Pocinho/LConn1 -- _CN_127205641_220000_CN_127205502_220000/LConn1 -- _CN_144432478_220000_CN_127205502_220000/LConn1 -- _CN_47895778_220000_CN_127205502_220000/LConn1
  _CN_144396420_220000_CN_127205502_220000/RConn2 -- T_127205502_220000_Subestação_de_Pocinho/LConn2 -- _CN_127205641_220000_CN_127205502_220000/LConn2 -- _CN_144432478_220000_CN_127205502_220000/LConn2 -- _CN_47895778_220000_CN_127205502_220000/LConn2
  _CN_144396420_220000_CN_127205502_220000/RConn3 -- T_127205502_220000_Subestação_de_Pocinho/LConn3 -- _CN_127205641_220000_CN_127205502_220000/LConn3 -- _CN_144432478_220000_CN_127205502_220000/LConn3 -- _CN_47895778_220000_CN_127205502_220000/LConn3 -- bus51/LConn1
  _CN_144396420_220000_CN_144396412_220000/RConn1 -- T_144396412_400000;220000_Subestação_de_Armamar/RConn1 -- L_144396412/LConn1
  _CN_144396420_220000_CN_144396412_220000/RConn2 -- T_144396412_400000;220000_Subestação_de_Armamar/RConn2 -- L_144396412/LConn2
  _CN_144396420_220000_CN_144396412_220000/RConn3 -- T_144396412_400000;220000_Subestação_de_Armamar/RConn3 -- L_144396412/LConn3 -- bus52/LConn1
  T_144396428_220000_/LConn1 -- _CN_144396420_220000_CN_144396428_220000/RConn1
  T_144396428_220000_/LConn2 -- _CN_144396420_220000_CN_144396428_220000/RConn2
  _CN_144396420_220000_CN_144396428_220000/RConn3 -- T_144396428_220000_/LConn3 -- bus53/LConn1
  T_127205641_220000_/LConn1 -- _CN_127205641_220000_CN_127205502_220000/RConn1
  T_127205641_220000_/LConn2 -- _CN_127205641_220000_CN_127205502_220000/RConn2
  _CN_127205641_220000_CN_127205502_220000/RConn3 -- T_127205641_220000_/LConn3 -- bus54/LConn1
  _CN_151162379_220000_CN_144545398_220000/LConn1 -- T_151162379_150000;60000_Subestação_de_Mourisca/LConn1 -- _CN_151162379_220000_CN_144374442_220000/LConn1 -- _CN_151162379_220000_CN_144439469_220000/LConn1 -- _CN_151162379_220000_CN_144374439_220000/RConn1
  _CN_151162379_220000_CN_144545398_220000/LConn2 -- T_151162379_150000;60000_Subestação_de_Mourisca/LConn2 -- _CN_151162379_220000_CN_144374442_220000/LConn2 -- _CN_151162379_220000_CN_144439469_220000/LConn2 -- _CN_151162379_220000_CN_144374439_220000/RConn2
  _CN_151162379_220000_CN_144545398_220000/LConn3 -- T_151162379_150000;60000_Subestação_de_Mourisca/LConn3 -- _CN_151162379_220000_CN_144374442_220000/LConn3 -- _CN_151162379_220000_CN_144439469_220000/LConn3 -- _CN_151162379_220000_CN_144374439_220000/RConn3 -- bus55/LConn1
  _CN_151162379_220000_CN_144545398_220000/RConn1 -- T_144545398_220000;60000_Subestação_de_Pereiros/LConn1 -- _CN_144545398_220000_CN_144584585_220000/LConn1 -- _CN_144545398_220000_CN_144545399_220000/LConn1 -- _CN_144545398_220000_CN_144584580_220000/LConn1 -- _CN_144545398_220000_CN_144564903_220000/LConn1 -- _CN_144545398_220000_CN_131715746_220000/LConn1
  _CN_151162379_220000_CN_144545398_220000/RConn2 -- T_144545398_220000;60000_Subestação_de_Pereiros/LConn2 -- _CN_144545398_220000_CN_144584585_220000/LConn2 -- _CN_144545398_220000_CN_144545399_220000/LConn2 -- _CN_144545398_220000_CN_144584580_220000/LConn2 -- _CN_144545398_220000_CN_144564903_220000/LConn2 -- _CN_144545398_220000_CN_131715746_220000/LConn2
  _CN_151162379_220000_CN_144545398_220000/RConn3 -- T_144545398_220000;60000_Subestação_de_Pereiros/LConn3 -- _CN_144545398_220000_CN_144584585_220000/LConn3 -- _CN_144545398_220000_CN_144545399_220000/LConn3 -- _CN_144545398_220000_CN_144584580_220000/LConn3 -- _CN_144545398_220000_CN_144564903_220000/LConn3 -- _CN_144545398_220000_CN_131715746_220000/LConn3 -- bus56/LConn1
  _CN_151162379_220000_CN_144374442_220000/RConn1 -- T_144374442_220000;60000_Subestação_de_Estarreja/LConn1 -- _CN_144374439_220000_CN_144374442_220000/RConn1 -- _CN_144374442_220000_CN_142658477_220000/LConn1 -- _CN_144374442_220000_CN_116944631_220000/LConn1
  _CN_151162379_220000_CN_144374442_220000/RConn2 -- T_144374442_220000;60000_Subestação_de_Estarreja/LConn2 -- _CN_144374439_220000_CN_144374442_220000/RConn2 -- _CN_144374442_220000_CN_142658477_220000/LConn2 -- _CN_144374442_220000_CN_116944631_220000/LConn2
  _CN_151162379_220000_CN_144374442_220000/RConn3 -- T_144374442_220000;60000_Subestação_de_Estarreja/LConn3 -- _CN_144374439_220000_CN_144374442_220000/RConn3 -- _CN_144374442_220000_CN_142658477_220000/LConn3 -- _CN_144374442_220000_CN_116944631_220000/LConn3 -- bus57/LConn1
  _CN_151162379_220000_CN_144439469_220000/RConn1 -- T_144439469_400000;220000;60000_Subestação_de_Paraimo/RConn1 -- L_144439469/LConn1
  _CN_151162379_220000_CN_144439469_220000/RConn2 -- T_144439469_400000;220000;60000_Subestação_de_Paraimo/RConn2 -- L_144439469/LConn2
  _CN_151162379_220000_CN_144439469_220000/RConn3 -- T_144439469_400000;220000;60000_Subestação_de_Paraimo/RConn3 -- L_144439469/LConn3 -- bus58/LConn1
  _CN_24636044_220000_CN_435865807_220000/LConn1 -- T_24636044_400000;220000;150000_Subestação_de_Fanhões/RConn1 -- _CN_24636044_220000_CN_151166980_220000/LConn1 -- _CN_24636044_220000_CN_144762180_220000/LConn1 -- _CN_24636044_220000_CN_24636062_220000/LConn1 -- _CN_24636044_220000_CN_144654759_220000/LConn1 -- _CN_24636044_220000_CN_151168335_220000/LConn1 -- _CN_24636044_220000_CN_144651478_220000/LConn1 -- _CN_24636044_220000_CN_131715746_220000/LConn1
  _CN_24636044_220000_CN_435865807_220000/LConn2 -- T_24636044_400000;220000;150000_Subestação_de_Fanhões/RConn2 -- _CN_24636044_220000_CN_151166980_220000/LConn2 -- _CN_24636044_220000_CN_144762180_220000/LConn2 -- _CN_24636044_220000_CN_24636062_220000/LConn2 -- _CN_24636044_220000_CN_144654759_220000/LConn2 -- _CN_24636044_220000_CN_151168335_220000/LConn2 -- _CN_24636044_220000_CN_144651478_220000/LConn2 -- _CN_24636044_220000_CN_131715746_220000/LConn2
  _CN_24636044_220000_CN_435865807_220000/LConn3 -- T_24636044_400000;220000;150000_Subestação_de_Fanhões/RConn3 -- _CN_24636044_220000_CN_151166980_220000/LConn3 -- bus59/LConn1 -- _CN_24636044_220000_CN_144762180_220000/LConn3 -- _CN_24636044_220000_CN_24636062_220000/LConn3 -- _CN_24636044_220000_CN_144654759_220000/LConn3 -- _CN_24636044_220000_CN_151168335_220000/LConn3 -- _CN_24636044_220000_CN_144651478_220000/LConn3 -- _CN_24636044_220000_CN_131715746_220000/LConn3
  _CN_24636044_220000_CN_435865807_220000/RConn1 -- T_435865807__/LConn1 -- _CN_435865807_220000_CN_131715746_220000/LConn1 -- _CN_435865807_220000_CN_144703168_220000/LConn1 -- _CN_435865807_220000_CN_144596347_220000/LConn1
  _CN_24636044_220000_CN_435865807_220000/RConn2 -- T_435865807__/LConn2 -- _CN_435865807_220000_CN_131715746_220000/LConn2 -- _CN_435865807_220000_CN_144703168_220000/LConn2 -- _CN_435865807_220000_CN_144596347_220000/LConn2
  _CN_24636044_220000_CN_435865807_220000/RConn3 -- T_435865807__/LConn3 -- _CN_435865807_220000_CN_131715746_220000/LConn3 -- _CN_435865807_220000_CN_144703168_220000/LConn3 -- _CN_435865807_220000_CN_144596347_220000/LConn3 -- bus60/LConn1
  _CN_24636044_220000_CN_144762180_220000/RConn1 -- T_144762180_220000_/LConn1 -- _CN_402947133_220000_CN_144762180_220000/LConn1
  _CN_24636044_220000_CN_144762180_220000/RConn2 -- T_144762180_220000_/LConn2 -- _CN_402947133_220000_CN_144762180_220000/LConn2
  _CN_24636044_220000_CN_144762180_220000/RConn3 -- T_144762180_220000_/LConn3 -- _CN_402947133_220000_CN_144762180_220000/LConn3 -- bus61/LConn1
  _CN_24636044_220000_CN_24636062_220000/RConn1 -- T_24636062_220000_/LConn1 -- _CN_24636062_220000_CN_183668286_220000/LConn1
  _CN_24636044_220000_CN_24636062_220000/RConn2 -- T_24636062_220000_/LConn2 -- _CN_24636062_220000_CN_183668286_220000/LConn2
  _CN_24636044_220000_CN_24636062_220000/RConn3 -- T_24636062_220000_/LConn3 -- _CN_24636062_220000_CN_183668286_220000/LConn3 -- bus62/LConn1
  T_144654759_220000_/LConn1 -- _CN_24636044_220000_CN_144654759_220000/RConn1
  T_144654759_220000_/LConn2 -- _CN_24636044_220000_CN_144654759_220000/RConn2
  _CN_24636044_220000_CN_144654759_220000/RConn3 -- T_144654759_220000_/LConn3 -- bus63/LConn1
  _CN_24636044_220000_CN_151168335_220000/RConn1 -- T_151168335_400000;220000;60000_/RConn1 -- _CN_183668286_220000_CN_151168335_220000/LConn1 -- L_151168335/LConn1
  _CN_24636044_220000_CN_151168335_220000/RConn2 -- T_151168335_400000;220000;60000_/RConn2 -- _CN_183668286_220000_CN_151168335_220000/LConn2 -- L_151168335/LConn2
  _CN_24636044_220000_CN_151168335_220000/RConn3 -- T_151168335_400000;220000;60000_/RConn3 -- _CN_183668286_220000_CN_151168335_220000/LConn3 -- L_151168335/LConn3 -- bus64/LConn1
  T_144651478_220000_/LConn1 -- _CN_24636044_220000_CN_144651478_220000/RConn1
  T_144651478_220000_/LConn2 -- _CN_24636044_220000_CN_144651478_220000/RConn2
  _CN_24636044_220000_CN_144651478_220000/RConn3 -- T_144651478_220000_/LConn3 -- bus65/LConn1
  _CN_24636044_220000_CN_131715746_220000/RConn1 -- T_131715746_400000_Subestação_de_Rio_Maior/RConn1 -- _CN_144545398_220000_CN_131715746_220000/RConn1 -- _CN_435865807_220000_CN_131715746_220000/RConn1 -- _CN_131715746_220000_CN_144564903_220000/LConn1 -- L_131715746/LConn1
  _CN_24636044_220000_CN_131715746_220000/RConn2 -- T_131715746_400000_Subestação_de_Rio_Maior/RConn2 -- _CN_144545398_220000_CN_131715746_220000/RConn2 -- _CN_435865807_220000_CN_131715746_220000/RConn2 -- _CN_131715746_220000_CN_144564903_220000/LConn2 -- L_131715746/LConn2
  _CN_24636044_220000_CN_131715746_220000/RConn3 -- T_131715746_400000_Subestação_de_Rio_Maior/RConn3 -- _CN_144545398_220000_CN_131715746_220000/RConn3 -- _CN_435865807_220000_CN_131715746_220000/RConn3 -- _CN_131715746_220000_CN_144564903_220000/LConn3 -- L_131715746/LConn3 -- bus66/LConn1
  T_151166980_220000_/LConn1 -- _CN_24636044_220000_CN_151166980_220000/RConn1
  T_151166980_220000_/LConn2 -- _CN_24636044_220000_CN_151166980_220000/RConn2
  _CN_24636044_220000_CN_151166980_220000/RConn3 -- T_151166980_220000_/LConn3 -- bus67/LConn1
  _CN_144545398_220000_CN_144584585_220000/RConn1 -- T_144584585_220000;60000_Subestação_de_Tábua/LConn1 -- _CN_144584585_220000_CN_137667702_220000/LConn1 -- _CN_144584580_220000_CN_144584585_220000/LConn1 -- _CN_144586949_220000_CN_144584585_220000/LConn1
  _CN_144545398_220000_CN_144584585_220000/RConn2 -- T_144584585_220000;60000_Subestação_de_Tábua/LConn2 -- _CN_144584585_220000_CN_137667702_220000/LConn2 -- _CN_144584580_220000_CN_144584585_220000/LConn2 -- _CN_144586949_220000_CN_144584585_220000/LConn2
  _CN_144545398_220000_CN_144584585_220000/RConn3 -- T_144584585_220000;60000_Subestação_de_Tábua/LConn3 -- _CN_144584585_220000_CN_137667702_220000/LConn3 -- bus68/LConn1 -- _CN_144584580_220000_CN_144584585_220000/LConn3 -- _CN_144586949_220000_CN_144584585_220000/LConn3
  T_144545399_220000_/LConn1 -- _CN_144545398_220000_CN_144545399_220000/RConn1
  T_144545399_220000_/LConn2 -- _CN_144545398_220000_CN_144545399_220000/RConn2
  _CN_144545398_220000_CN_144545399_220000/RConn3 -- T_144545399_220000_/LConn3 -- bus69/LConn1
  _CN_144545398_220000_CN_144584580_220000/RConn1 -- T_144584580_220000_Subestação_de_Penela/LConn1 -- _CN_144584580_220000_CN_144584585_220000/RConn1 -- _CN_144584580_220000_CN_144588414_220000/LConn1
  _CN_144545398_220000_CN_144584580_220000/RConn2 -- T_144584580_220000_Subestação_de_Penela/LConn2 -- _CN_144584580_220000_CN_144584585_220000/RConn2 -- _CN_144584580_220000_CN_144588414_220000/LConn2
  _CN_144545398_220000_CN_144584580_220000/RConn3 -- T_144584580_220000_Subestação_de_Penela/LConn3 -- _CN_144584580_220000_CN_144584585_220000/RConn3 -- bus70/LConn1 -- _CN_144584580_220000_CN_144588414_220000/LConn3
  _CN_144545398_220000_CN_144564903_220000/RConn1 -- T_144564903_400000;220000;150000_Subestação_do_Celeiro/RConn1 -- _CN_131715746_220000_CN_144564903_220000/RConn1 -- L_144564903/LConn1
  _CN_144545398_220000_CN_144564903_220000/RConn2 -- T_144564903_400000;220000;150000_Subestação_do_Celeiro/RConn2 -- _CN_131715746_220000_CN_144564903_220000/RConn2 -- L_144564903/LConn2
  _CN_144545398_220000_CN_144564903_220000/RConn3 -- T_144564903_400000;220000;150000_Subestação_do_Celeiro/RConn3 -- _CN_131715746_220000_CN_144564903_220000/RConn3 -- L_144564903/LConn3 -- bus71/LConn1
  T_144703168_220000_Subestação_de_Seixal/LConn1 -- _CN_435865807_220000_CN_144703168_220000/RConn1
  T_144703168_220000_Subestação_de_Seixal/LConn2 -- _CN_435865807_220000_CN_144703168_220000/RConn2
  _CN_435865807_220000_CN_144703168_220000/RConn3 -- T_144703168_220000_Subestação_de_Seixal/LConn3 -- bus72/LConn1
  _CN_435865807_220000_CN_144596347_220000/RConn1 -- T_144596347_220000_Subestação_de_Santarém/LConn1 -- _CN_144588414_220000_CN_144596347_220000/LConn1
  _CN_435865807_220000_CN_144596347_220000/RConn2 -- T_144596347_220000_Subestação_de_Santarém/LConn2 -- _CN_144588414_220000_CN_144596347_220000/LConn2
  _CN_435865807_220000_CN_144596347_220000/RConn3 -- T_144596347_220000_Subestação_de_Santarém/LConn3 -- _CN_144588414_220000_CN_144596347_220000/LConn3 -- bus73/LConn1
  T_151111218_220000_/LConn1 -- _CN_151111218_220000_CN_144377301_220000/LConn1
  T_151111218_220000_/LConn2 -- _CN_151111218_220000_CN_144377301_220000/LConn2
  _CN_151111218_220000_CN_144377301_220000/LConn3 -- T_151111218_220000_/LConn3 -- bus74/LConn1
  _CN_151111218_220000_CN_144377301_220000/RConn1 -- T_144377301_220000;60000_Sub_Estação_de_Custóias/LConn1 -- _CN_142182853_220000_CN_144377301_220000/LConn1
  _CN_151111218_220000_CN_144377301_220000/RConn2 -- T_144377301_220000;60000_Sub_Estação_de_Custóias/LConn2 -- _CN_142182853_220000_CN_144377301_220000/LConn2
  _CN_151111218_220000_CN_144377301_220000/RConn3 -- T_144377301_220000;60000_Sub_Estação_de_Custóias/LConn3 -- _CN_142182853_220000_CN_144377301_220000/LConn3 -- bus75/LConn1
  _CN_127205653_220000_CN_144374439_220000/RConn1 -- T_127205653_220000_/LConn1 -- _CN_127205653_220000_CN_144387430_220000/LConn1 -- _CN_127205653_220000_CN_144385735_220000/LConn1 -- _CN_127205653_220000_CN_144385734_220000/LConn1
  _CN_127205653_220000_CN_144374439_220000/RConn2 -- T_127205653_220000_/LConn2 -- _CN_127205653_220000_CN_144387430_220000/LConn2 -- _CN_127205653_220000_CN_144385735_220000/LConn2 -- _CN_127205653_220000_CN_144385734_220000/LConn2
  _CN_127205653_220000_CN_144374439_220000/RConn3 -- T_127205653_220000_/LConn3 -- _CN_127205653_220000_CN_144387430_220000/LConn3 -- _CN_127205653_220000_CN_144385735_220000/LConn3 -- _CN_127205653_220000_CN_144385734_220000/LConn3 -- bus76/LConn1
  T_144387430_220000_/LConn1 -- _CN_127205653_220000_CN_144387430_220000/RConn1
  T_144387430_220000_/LConn2 -- _CN_127205653_220000_CN_144387430_220000/RConn2
  _CN_127205653_220000_CN_144387430_220000/RConn3 -- T_144387430_220000_/LConn3 -- bus77/LConn1
  _CN_127205653_220000_CN_144385735_220000/RConn1 -- T_144385735_220000_/LConn1 -- _CN_144385734_220000_CN_144385735_220000/LConn1
  _CN_127205653_220000_CN_144385735_220000/RConn2 -- T_144385735_220000_/LConn2 -- _CN_144385734_220000_CN_144385735_220000/LConn2
  _CN_127205653_220000_CN_144385735_220000/RConn3 -- T_144385735_220000_/LConn3 -- _CN_144385734_220000_CN_144385735_220000/LConn3 -- bus78/LConn1
  _CN_127205653_220000_CN_144385734_220000/RConn1 -- T_144385734_400000;220000_Subestação_de_Lagoaça/RConn1 -- _CN_144385734_220000_CN_144385735_220000/RConn1 -- L_144385734/LConn1 -- _CN_144386243_220000_CN_144385734_220000/LConn1
  _CN_127205653_220000_CN_144385734_220000/RConn2 -- T_144385734_400000;220000_Subestação_de_Lagoaça/RConn2 -- _CN_144385734_220000_CN_144385735_220000/RConn2 -- L_144385734/LConn2 -- _CN_144386243_220000_CN_144385734_220000/LConn2
  _CN_127205653_220000_CN_144385734_220000/RConn3 -- T_144385734_400000;220000_Subestação_de_Lagoaça/RConn3 -- _CN_144385734_220000_CN_144385735_220000/RConn3 -- L_144385734/LConn3 -- bus79/LConn1 -- _CN_144386243_220000_CN_144385734_220000/LConn3
  _CN_144584580_220000_CN_144588414_220000/RConn1 -- T_144588414_220000;60000_Subestação_REN_Zêzere/LConn1 -- _CN_144588414_220000_CN_144596347_220000/RConn1
  _CN_144584580_220000_CN_144588414_220000/RConn2 -- T_144588414_220000;60000_Subestação_REN_Zêzere/LConn2 -- _CN_144588414_220000_CN_144596347_220000/RConn2
  _CN_144584580_220000_CN_144588414_220000/RConn3 -- T_144588414_220000;60000_Subestação_REN_Zêzere/LConn3 -- _CN_144588414_220000_CN_144596347_220000/RConn3 -- bus80/LConn1
  _CN_24636062_220000_CN_183668286_220000/RConn1 -- T_183668286_220000;60000_Subestação_de_Sete_Rios/LConn1 -- _CN_183668286_220000_CN_151168335_220000/RConn1
  _CN_24636062_220000_CN_183668286_220000/RConn2 -- T_183668286_220000;60000_Subestação_de_Sete_Rios/LConn2 -- _CN_183668286_220000_CN_151168335_220000/RConn2
  _CN_24636062_220000_CN_183668286_220000/RConn3 -- T_183668286_220000;60000_Subestação_de_Sete_Rios/LConn3 -- _CN_183668286_220000_CN_151168335_220000/RConn3 -- bus81/LConn1
  T_144586949_220000_/LConn1 -- _CN_144586949_220000_CN_144584585_220000/RConn1
  T_144586949_220000_/LConn2 -- _CN_144586949_220000_CN_144584585_220000/RConn2
  _CN_144586949_220000_CN_144584585_220000/RConn3 -- T_144586949_220000_/LConn3 -- bus82/LConn1
  _CN_144374442_220000_CN_142658477_220000/RConn1 -- T_142658477_220000_/LConn1 -- _CN_142658477_220000_CN_124722161_220000/RConn1
  _CN_144374442_220000_CN_142658477_220000/RConn2 -- T_142658477_220000_/LConn2 -- _CN_142658477_220000_CN_124722161_220000/RConn2
  _CN_144374442_220000_CN_142658477_220000/RConn3 -- T_142658477_220000_/LConn3 -- _CN_142658477_220000_CN_124722161_220000/RConn3 -- bus83/LConn1
  T_116944631_220000;60000_Subestação_de_Canelas/LConn1 -- _CN_144374442_220000_CN_116944631_220000/RConn1
  T_116944631_220000;60000_Subestação_de_Canelas/LConn2 -- _CN_144374442_220000_CN_116944631_220000/RConn2
  _CN_144374442_220000_CN_116944631_220000/RConn3 -- T_116944631_220000;60000_Subestação_de_Canelas/LConn3 -- bus84/LConn1
  _CN_47911346_220000_CN_47895778_220000/LConn1 -- T_47911346_400000_/RConn1 -- L_47911346/LConn1
  _CN_47911346_220000_CN_47895778_220000/LConn2 -- T_47911346_400000_/RConn2 -- L_47911346/LConn2
  _CN_47911346_220000_CN_47895778_220000/LConn3 -- T_47911346_400000_/RConn3 -- L_47911346/LConn3 -- bus85/LConn1
  _CN_47911346_220000_CN_47895778_220000/RConn1 -- T_47895778_220000_/LConn1 -- _CN_47895778_220000_CN_127205502_220000/RConn1
  _CN_47911346_220000_CN_47895778_220000/RConn2 -- T_47895778_220000_/LConn2 -- _CN_47895778_220000_CN_127205502_220000/RConn2
  _CN_47911346_220000_CN_47895778_220000/RConn3 -- T_47895778_220000_/LConn3 -- _CN_47895778_220000_CN_127205502_220000/RConn3 -- bus86/LConn1
  _CN_144584585_220000_CN_137667702_220000/RConn1 -- T_137667702_220000;60000_Subestação_de_Vila_Chã/LConn1 -- _CN_144433994_220000_CN_137667702_220000/LConn1
  _CN_144584585_220000_CN_137667702_220000/RConn2 -- T_137667702_220000;60000_Subestação_de_Vila_Chã/LConn2 -- _CN_144433994_220000_CN_137667702_220000/LConn2
  _CN_144584585_220000_CN_137667702_220000/RConn3 -- T_137667702_220000;60000_Subestação_de_Vila_Chã/LConn3 -- _CN_144433994_220000_CN_137667702_220000/LConn3 -- bus87/LConn1
  T_144552378_220000;150000;60000_/LConn1 -- _CN_144552378_220000_CN_144432489_220000/LConn1
  T_144552378_220000;150000;60000_/LConn2 -- _CN_144552378_220000_CN_144432489_220000/LConn2
  _CN_144552378_220000_CN_144432489_220000/LConn3 -- T_144552378_220000;150000;60000_/LConn3 -- bus88/LConn1
  _CN_144552378_220000_CN_144432489_220000/RConn1 -- T_144432489_220000_Subestação_do_Ferro/LConn1 -- _CN_121159140_220000_CN_144432489_220000/LConn1 -- _CN_144432478_220000_CN_144432489_220000/LConn1
  _CN_144552378_220000_CN_144432489_220000/RConn2 -- T_144432489_220000_Subestação_do_Ferro/LConn2 -- _CN_121159140_220000_CN_144432489_220000/LConn2 -- _CN_144432478_220000_CN_144432489_220000/LConn2
  _CN_144552378_220000_CN_144432489_220000/RConn3 -- T_144432489_220000_Subestação_do_Ferro/LConn3 -- _CN_121159140_220000_CN_144432489_220000/LConn3 -- bus89/LConn1 -- _CN_144432478_220000_CN_144432489_220000/LConn3
  T_402947133_220000_Subestação_de_Sacavém/LConn1 -- _CN_402947133_220000_CN_144762180_220000/RConn1
  T_402947133_220000_Subestação_de_Sacavém/LConn2 -- _CN_402947133_220000_CN_144762180_220000/RConn2
  _CN_402947133_220000_CN_144762180_220000/RConn3 -- T_402947133_220000_Subestação_de_Sacavém/LConn3 -- bus90/LConn1
  T_144386243_220000_/LConn1 -- _CN_144386243_220000_CN_144385734_220000/RConn1
  T_144386243_220000_/LConn2 -- _CN_144386243_220000_CN_144385734_220000/RConn2
  _CN_144386243_220000_CN_144385734_220000/RConn3 -- T_144386243_220000_/LConn3 -- bus91/LConn1
  _CN_142182853_220000_CN_144377301_220000/RConn1 -- T_142182853_220000;150000;60000_Subestação_de_Vermoim/LConn1 -- _CN_142182853_220000_CN_124722161_220000/RConn1
  _CN_142182853_220000_CN_144377301_220000/RConn2 -- T_142182853_220000;150000;60000_Subestação_de_Vermoim/LConn2 -- _CN_142182853_220000_CN_124722161_220000/RConn2
  _CN_142182853_220000_CN_144377301_220000/RConn3 -- T_142182853_220000;150000;60000_Subestação_de_Vermoim/LConn3 -- _CN_142182853_220000_CN_124722161_220000/RConn3 -- bus92/LConn1
  _CN_144433994_220000_CN_137667702_220000/RConn1 -- T_144433994_220000_/LConn1 -- _CN_144433994_220000_CN_144432478_220000/LConn1
  _CN_144433994_220000_CN_137667702_220000/RConn2 -- T_144433994_220000_/LConn2 -- _CN_144433994_220000_CN_144432478_220000/LConn2
  _CN_144433994_220000_CN_137667702_220000/RConn3 -- T_144433994_220000_/LConn3 -- _CN_144433994_220000_CN_144432478_220000/LConn3 -- bus93/LConn1
  _CN_144433994_220000_CN_144432478_220000/RConn1 -- T_144432478_220000_/LConn1 -- _CN_144432478_220000_CN_144432485_220000/LConn1 -- _CN_144432478_220000_CN_144432489_220000/RConn1 -- _CN_144432478_220000_CN_127205502_220000/RConn1
  _CN_144433994_220000_CN_144432478_220000/RConn2 -- T_144432478_220000_/LConn2 -- _CN_144432478_220000_CN_144432485_220000/LConn2 -- _CN_144432478_220000_CN_144432489_220000/RConn2 -- _CN_144432478_220000_CN_127205502_220000/RConn2
  _CN_144433994_220000_CN_144432478_220000/RConn3 -- T_144432478_220000_/LConn3 -- _CN_144432478_220000_CN_144432485_220000/LConn3 -- _CN_144432478_220000_CN_144432489_220000/RConn3 -- bus94/LConn1 -- _CN_144432478_220000_CN_127205502_220000/RConn3
  T_144432485_220000_Subestação_de_Sobral/LConn1 -- _CN_144432478_220000_CN_144432485_220000/RConn1
  T_144432485_220000_Subestação_de_Sobral/LConn2 -- _CN_144432478_220000_CN_144432485_220000/RConn2
  _CN_144432478_220000_CN_144432485_220000/RConn3 -- T_144432485_220000_Subestação_de_Sobral/LConn3 -- bus95/LConn1
  T_121159140_220000;60000_/LConn1 -- _CN_121159140_220000_CN_144432489_220000/RConn1
  T_121159140_220000;60000_/LConn2 -- _CN_121159140_220000_CN_144432489_220000/RConn2
  _CN_121159140_220000_CN_144432489_220000/RConn3 -- T_121159140_220000;60000_/LConn3 -- bus96/LConn1
  T_144601080__/LConn1 -- _CN_144601080_220000_CN_144599061_220000/LConn1
  T_144601080__/LConn2 -- _CN_144601080_220000_CN_144599061_220000/LConn2
  _CN_144601080_220000_CN_144599061_220000/LConn3 -- T_144601080__/LConn3 -- bus97/LConn1
  _CN_144601080_220000_CN_144599061_220000/RConn1 -- T_144599061_400000_/RConn1 -- L_144599061/LConn1
  _CN_144601080_220000_CN_144599061_220000/RConn2 -- T_144599061_400000_/RConn2 -- L_144599061/LConn2
  _CN_144601080_220000_CN_144599061_220000/RConn3 -- T_144599061_400000_/RConn3 -- L_144599061/LConn3 -- bus98/LConn1
  _CN_144622215_400000_CN_144635505_400000/LConn1 -- T_144622215_400000;150000_Subestação_de_Sines/LConn1 -- _CN_144622215_400000_CN_129055610_400000/LConn1 -- _CN_144622215_400000_CN_109866595_150000/RConn1
  _CN_144622215_400000_CN_144635505_400000/LConn2 -- T_144622215_400000;150000_Subestação_de_Sines/LConn2 -- _CN_144622215_400000_CN_129055610_400000/LConn2 -- _CN_144622215_400000_CN_109866595_150000/RConn2
  _CN_144622215_400000_CN_144635505_400000/LConn3 -- T_144622215_400000;150000_Subestação_de_Sines/LConn3 -- _CN_144622215_400000_CN_129055610_400000/LConn3 -- _CN_144622215_400000_CN_109866595_150000/RConn3 -- bus99/LConn1
  _CN_144622215_400000_CN_144635505_400000/RConn1 -- T_144635505_400000;150000_Subestação_de_Ferreira_do_Alentejo/LConn1 -- _CN_144639174_400000_CN_144635505_400000/LConn1
  _CN_144622215_400000_CN_144635505_400000/RConn2 -- T_144635505_400000;150000_Subestação_de_Ferreira_do_Alentejo/LConn2 -- _CN_144639174_400000_CN_144635505_400000/LConn2
  _CN_144622215_400000_CN_144635505_400000/RConn3 -- T_144635505_400000;150000_Subestação_de_Ferreira_do_Alentejo/LConn3 -- _CN_144639174_400000_CN_144635505_400000/LConn3 -- bus100/LConn1
  _CN_144622215_400000_CN_129055610_400000/RConn1 -- T_129055610_400000;150000_Subestação_de_Palmela/LConn1 -- _CN_24636044_400000_CN_129055610_400000/LConn1 -- _CN_144564903_400000_CN_129055610_400000/LConn1 -- _CN_144708196_400000_CN_129055610_400000/LConn1
  _CN_144622215_400000_CN_129055610_400000/RConn2 -- T_129055610_400000;150000_Subestação_de_Palmela/LConn2 -- _CN_24636044_400000_CN_129055610_400000/LConn2 -- _CN_144564903_400000_CN_129055610_400000/LConn2 -- _CN_144708196_400000_CN_129055610_400000/LConn2
  _CN_144622215_400000_CN_129055610_400000/RConn3 -- T_129055610_400000;150000_Subestação_de_Palmela/LConn3 -- _CN_24636044_400000_CN_129055610_400000/LConn3 -- _CN_144564903_400000_CN_129055610_400000/LConn3 -- _CN_144708196_400000_CN_129055610_400000/LConn3 -- bus101/LConn1
  _CN_24636044_400000_CN_144608818_400000/LConn1 -- T_24636044_400000;220000;150000_Subestação_de_Fanhões/LConn1 -- _CN_24636044_400000_CN_129055610_400000/RConn1 -- _CN_24636044_400000_CN_151168335_400000/LConn1 -- _CN_24636044_400000_CN_131715746_400000/LConn1
  _CN_24636044_400000_CN_144608818_400000/LConn2 -- T_24636044_400000;220000;150000_Subestação_de_Fanhões/LConn2 -- _CN_24636044_400000_CN_129055610_400000/RConn2 -- _CN_24636044_400000_CN_151168335_400000/LConn2 -- _CN_24636044_400000_CN_131715746_400000/LConn2
  _CN_24636044_400000_CN_144608818_400000/LConn3 -- T_24636044_400000;220000;150000_Subestação_de_Fanhões/LConn3 -- _CN_24636044_400000_CN_129055610_400000/RConn3 -- bus102/LConn1 -- _CN_24636044_400000_CN_151168335_400000/LConn3 -- _CN_24636044_400000_CN_131715746_400000/LConn3
  _CN_24636044_400000_CN_144608818_400000/RConn1 -- T_144608818_400000_/LConn1 -- _CN_144564903_400000_CN_144608818_400000/LConn1 -- _CN_144608818_400000_CN_138358013_400000/LConn1
  _CN_24636044_400000_CN_144608818_400000/RConn2 -- T_144608818_400000_/LConn2 -- _CN_144564903_400000_CN_144608818_400000/LConn2 -- _CN_144608818_400000_CN_138358013_400000/LConn2
  _CN_24636044_400000_CN_144608818_400000/RConn3 -- T_144608818_400000_/LConn3 -- _CN_144564903_400000_CN_144608818_400000/LConn3 -- _CN_144608818_400000_CN_138358013_400000/LConn3 -- bus103/LConn1
  T_151168335_400000;220000;60000_/LConn1 -- _CN_24636044_400000_CN_151168335_400000/RConn1
  T_151168335_400000;220000;60000_/LConn2 -- _CN_24636044_400000_CN_151168335_400000/RConn2
  _CN_24636044_400000_CN_151168335_400000/RConn3 -- T_151168335_400000;220000;60000_/LConn3 -- bus104/LConn1
  _CN_24636044_400000_CN_131715746_400000/RConn1 -- T_131715746_400000_Subestação_de_Rio_Maior/LConn1 -- _CN_131715746_400000_CN_144573746_400000/LConn1 -- _CN_131715746_400000_CN_144554435_400000/LConn1 -- _CN_131715746_400000_CN_124722161_400000/LConn1
  _CN_24636044_400000_CN_131715746_400000/RConn2 -- T_131715746_400000_Subestação_de_Rio_Maior/LConn2 -- _CN_131715746_400000_CN_144573746_400000/LConn2 -- _CN_131715746_400000_CN_144554435_400000/LConn2 -- _CN_131715746_400000_CN_124722161_400000/LConn2
  _CN_24636044_400000_CN_131715746_400000/RConn3 -- T_131715746_400000_Subestação_de_Rio_Maior/LConn3 -- _CN_131715746_400000_CN_144573746_400000/LConn3 -- _CN_131715746_400000_CN_144554435_400000/LConn3 -- _CN_131715746_400000_CN_124722161_400000/LConn3 -- bus105/LConn1
  _CN_151162388_400000_CN_144564903_400000/LConn1 -- T_151162388_400000_/LConn1 -- _CN_151162388_400000_CN_151162382_400000/LConn1
  _CN_151162388_400000_CN_144564903_400000/LConn2 -- T_151162388_400000_/LConn2 -- _CN_151162388_400000_CN_151162382_400000/LConn2
  _CN_151162388_400000_CN_144564903_400000/LConn3 -- T_151162388_400000_/LConn3 -- _CN_151162388_400000_CN_151162382_400000/LConn3 -- bus106/LConn1
  _CN_151162388_400000_CN_144564903_400000/RConn1 -- T_144564903_400000;220000;150000_Subestação_do_Celeiro/LConn1 -- _CN_144564903_400000_CN_144573746_400000/LConn1 -- _CN_144564903_400000_CN_124722161_400000/LConn1 -- _CN_144564903_400000_CN_144439469_400000/LConn1 -- _CN_144564903_400000_CN_129055610_400000/RConn1 -- _CN_144564903_400000_CN_144608818_400000/RConn1
  _CN_151162388_400000_CN_144564903_400000/RConn2 -- T_144564903_400000;220000;150000_Subestação_do_Celeiro/LConn2 -- _CN_144564903_400000_CN_144573746_400000/LConn2 -- _CN_144564903_400000_CN_124722161_400000/LConn2 -- _CN_144564903_400000_CN_144439469_400000/LConn2 -- _CN_144564903_400000_CN_129055610_400000/RConn2 -- _CN_144564903_400000_CN_144608818_400000/RConn2
  _CN_151162388_400000_CN_144564903_400000/RConn3 -- T_144564903_400000;220000;150000_Subestação_do_Celeiro/LConn3 -- _CN_144564903_400000_CN_144573746_400000/LConn3 -- _CN_144564903_400000_CN_124722161_400000/LConn3 -- _CN_144564903_400000_CN_144439469_400000/LConn3 -- _CN_144564903_400000_CN_129055610_400000/RConn3 -- _CN_144564903_400000_CN_144608818_400000/RConn3 -- bus107/LConn1
  G_151162382_Central_de_Ciclo_Combinado_de_Lares/RConn1 -- _CN_151162388_400000_CN_151162382_400000/RConn1
  G_151162382_Central_de_Ciclo_Combinado_de_Lares/RConn2 -- _CN_151162388_400000_CN_151162382_400000/RConn2
  _CN_151162388_400000_CN_151162382_400000/RConn3 -- G_151162382_Central_de_Ciclo_Combinado_de_Lares/RConn3 -- bus108/LConn1
  _CN_144599061_400000_CN_84526032_400000/LConn1 -- T_144599061_400000_/LConn1 -- _CN_144599061_400000_CN_144573746_400000/LConn1
  _CN_144599061_400000_CN_84526032_400000/LConn2 -- T_144599061_400000_/LConn2 -- _CN_144599061_400000_CN_144573746_400000/LConn2
  _CN_144599061_400000_CN_84526032_400000/LConn3 -- T_144599061_400000_/LConn3 -- _CN_144599061_400000_CN_144573746_400000/LConn3 -- bus109/LConn1
  T_84526032_400000_/LConn1 -- _CN_144599061_400000_CN_84526032_400000/RConn1
  T_84526032_400000_/LConn2 -- _CN_144599061_400000_CN_84526032_400000/RConn2
  _CN_144599061_400000_CN_84526032_400000/RConn3 -- T_84526032_400000_/LConn3 -- bus110/LConn1
  _CN_144599061_400000_CN_144573746_400000/RConn1 -- T_144573746_400000_/LConn1 -- _CN_131715746_400000_CN_144573746_400000/RConn1 -- _CN_144564903_400000_CN_144573746_400000/RConn1
  _CN_144599061_400000_CN_144573746_400000/RConn2 -- T_144573746_400000_/LConn2 -- _CN_131715746_400000_CN_144573746_400000/RConn2 -- _CN_144564903_400000_CN_144573746_400000/RConn2
  _CN_144599061_400000_CN_144573746_400000/RConn3 -- T_144573746_400000_/LConn3 -- _CN_131715746_400000_CN_144573746_400000/RConn3 -- _CN_144564903_400000_CN_144573746_400000/RConn3 -- bus111/LConn1
  T_144554435_400000_Subestação_de_Lavos/LConn1 -- _CN_131715746_400000_CN_144554435_400000/RConn1
  T_144554435_400000_Subestação_de_Lavos/LConn2 -- _CN_131715746_400000_CN_144554435_400000/RConn2
  _CN_131715746_400000_CN_144554435_400000/RConn3 -- T_144554435_400000_Subestação_de_Lavos/LConn3 -- bus112/LConn1
  _CN_131715746_400000_CN_124722161_400000/RConn1 -- T_124722161_400000;220000;60000_Subestação_de_Recarei/LConn1 -- _CN_144564903_400000_CN_124722161_400000/RConn1 -- _CN_132865612_400000_CN_124722161_400000/LConn1
  _CN_131715746_400000_CN_124722161_400000/RConn2 -- T_124722161_400000;220000;60000_Subestação_de_Recarei/LConn2 -- _CN_144564903_400000_CN_124722161_400000/RConn2 -- _CN_132865612_400000_CN_124722161_400000/LConn2
  _CN_131715746_400000_CN_124722161_400000/RConn3 -- T_124722161_400000;220000;60000_Subestação_de_Recarei/LConn3 -- _CN_144564903_400000_CN_124722161_400000/RConn3 -- _CN_132865612_400000_CN_124722161_400000/LConn3 -- bus113/LConn1
  _CN_144385734_400000_CN_144396412_400000/LConn1 -- T_144385734_400000;220000_Subestação_de_Lagoaça/LConn1 -- _CN_144385734_400000_CN_47911346_400000/LConn1
  _CN_144385734_400000_CN_144396412_400000/LConn2 -- T_144385734_400000;220000_Subestação_de_Lagoaça/LConn2 -- _CN_144385734_400000_CN_47911346_400000/LConn2
  _CN_144385734_400000_CN_144396412_400000/LConn3 -- T_144385734_400000;220000_Subestação_de_Lagoaça/LConn3 -- _CN_144385734_400000_CN_47911346_400000/LConn3 -- bus114/LConn1
  _CN_144385734_400000_CN_144396412_400000/RConn1 -- T_144396412_400000;220000_Subestação_de_Armamar/LConn1 -- _CN_144439472_400000_CN_144396412_400000/LConn1
  _CN_144385734_400000_CN_144396412_400000/RConn2 -- T_144396412_400000;220000_Subestação_de_Armamar/LConn2 -- _CN_144439472_400000_CN_144396412_400000/LConn2
  _CN_144385734_400000_CN_144396412_400000/RConn3 -- T_144396412_400000;220000_Subestação_de_Armamar/LConn3 -- _CN_144439472_400000_CN_144396412_400000/LConn3 -- bus115/LConn1
  _CN_144385734_400000_CN_47911346_400000/RConn1 -- T_47911346_400000_/LConn1 -- _CN_47911346_400000_CN_144327157_400000/LConn1
  _CN_144385734_400000_CN_47911346_400000/RConn2 -- T_47911346_400000_/LConn2 -- _CN_47911346_400000_CN_144327157_400000/LConn2
  _CN_144385734_400000_CN_47911346_400000/RConn3 -- T_47911346_400000_/LConn3 -- _CN_47911346_400000_CN_144327157_400000/LConn3 -- bus116/LConn1
  _CN_144564903_400000_CN_144439469_400000/RConn1 -- T_144439469_400000;220000;60000_Subestação_de_Paraimo/LConn1 -- _CN_144439469_400000_CN_144439472_400000/LConn1
  _CN_144564903_400000_CN_144439469_400000/RConn2 -- T_144439469_400000;220000;60000_Subestação_de_Paraimo/LConn2 -- _CN_144439469_400000_CN_144439472_400000/LConn2
  _CN_144564903_400000_CN_144439469_400000/RConn3 -- T_144439469_400000;220000;60000_Subestação_de_Paraimo/LConn3 -- _CN_144439469_400000_CN_144439472_400000/LConn3 -- bus117/LConn1
  _CN_144439469_400000_CN_144439472_400000/RConn1 -- T_144439472_220000_/LConn1 -- _CN_144439472_400000_CN_144396412_400000/RConn1
  _CN_144439469_400000_CN_144439472_400000/RConn2 -- T_144439472_220000_/LConn2 -- _CN_144439472_400000_CN_144396412_400000/RConn2
  _CN_144439469_400000_CN_144439472_400000/RConn3 -- T_144439472_220000_/LConn3 -- _CN_144439472_400000_CN_144396412_400000/RConn3 -- bus118/LConn1
  T_144639174_400000;60000_Subestação_de_Alqueva/LConn1 -- _CN_144639174_400000_CN_144635505_400000/RConn1
  T_144639174_400000;60000_Subestação_de_Alqueva/LConn2 -- _CN_144639174_400000_CN_144635505_400000/RConn2
  _CN_144639174_400000_CN_144635505_400000/RConn3 -- T_144639174_400000;60000_Subestação_de_Alqueva/LConn3 -- bus119/LConn1
  T_135457228_400000_/LConn1 -- _CN_135457228_400000_CN_135457230_400000/LConn1
  T_135457228_400000_/LConn2 -- _CN_135457228_400000_CN_135457230_400000/LConn2
  _CN_135457228_400000_CN_135457230_400000/LConn3 -- T_135457228_400000_/LConn3 -- bus120/LConn1
  _CN_135457228_400000_CN_135457230_400000/RConn1 -- T_135457230_400000_/LConn1 -- _CN_132865612_400000_CN_135457230_400000/LConn1
  _CN_135457228_400000_CN_135457230_400000/RConn2 -- T_135457230_400000_/LConn2 -- _CN_132865612_400000_CN_135457230_400000/LConn2
  _CN_135457228_400000_CN_135457230_400000/RConn3 -- T_135457230_400000_/LConn3 -- _CN_132865612_400000_CN_135457230_400000/LConn3 -- bus121/LConn1
  _CN_132865612_400000_CN_135457230_400000/RConn1 -- T_132865612_400000;150000;60000_Subestação_de_Riba_de_Ave/LConn1 -- _CN_132865612_400000_CN_124722161_400000/RConn1 -- _CN_132865612_400000_CN_151061884_400000/LConn1
  _CN_132865612_400000_CN_135457230_400000/RConn2 -- T_132865612_400000;150000;60000_Subestação_de_Riba_de_Ave/LConn2 -- _CN_132865612_400000_CN_124722161_400000/RConn2 -- _CN_132865612_400000_CN_151061884_400000/LConn2
  _CN_132865612_400000_CN_135457230_400000/RConn3 -- T_132865612_400000;150000;60000_Subestação_de_Riba_de_Ave/LConn3 -- _CN_132865612_400000_CN_124722161_400000/RConn3 -- _CN_132865612_400000_CN_151061884_400000/LConn3 -- bus122/LConn1
  T_151061884_400000;15000_Subestação_de_Pedralva/LConn1 -- _CN_132865612_400000_CN_151061884_400000/RConn1
  T_151061884_400000;15000_Subestação_de_Pedralva/LConn2 -- _CN_132865612_400000_CN_151061884_400000/RConn2
  _CN_132865612_400000_CN_151061884_400000/RConn3 -- T_151061884_400000;15000_Subestação_de_Pedralva/LConn3 -- bus123/LConn1
  G_138358013_Central_Termoeléctrica_do_Ribatejo/RConn1 -- _CN_144608818_400000_CN_138358013_400000/RConn1
  G_138358013_Central_Termoeléctrica_do_Ribatejo/RConn2 -- _CN_144608818_400000_CN_138358013_400000/RConn2
  _CN_144608818_400000_CN_138358013_400000/RConn3 -- G_138358013_Central_Termoeléctrica_do_Ribatejo/RConn3 -- bus124/LConn1
  T_144708196_400000_/LConn1 -- _CN_144708196_400000_CN_129055610_400000/RConn1
  T_144708196_400000_/LConn2 -- _CN_144708196_400000_CN_129055610_400000/RConn2
  _CN_144708196_400000_CN_129055610_400000/RConn3 -- T_144708196_400000_/LConn3 -- bus125/LConn1
  T_144327157_400000;220000_Subestación_de_Villarino/LConn1 -- _CN_47911346_400000_CN_144327157_400000/RConn1
  T_144327157_400000;220000_Subestación_de_Villarino/LConn2 -- _CN_47911346_400000_CN_144327157_400000/RConn2
  _CN_47911346_400000_CN_144327157_400000/RConn3 -- T_144327157_400000;220000_Subestación_de_Villarino/LConn3 -- bus126/LConn1
  T_163204230_150000_Subestação_de_Neves_Corvo/RConn1 -- L_163204230/LConn1
  T_163204230_150000_Subestação_de_Neves_Corvo/RConn2 -- L_163204230/LConn2
  L_163204230/LConn3 -- T_163204230_150000_Subestação_de_Neves_Corvo/RConn3 -- bus127/LConn1
  T_115732510_150000_Subestação_de_Ourique/RConn1 -- L_115732510/LConn1
  T_115732510_150000_Subestação_de_Ourique/RConn2 -- L_115732510/LConn2
  L_115732510/LConn3 -- T_115732510_150000_Subestação_de_Ourique/RConn3 -- bus128/LConn1
  T_163194137_400000;150000_Subestação_de_Porto_de_Lagos/RConn1 -- L_163194137/LConn1
  T_163194137_400000;150000_Subestação_de_Porto_de_Lagos/RConn2 -- L_163194137/LConn2
  L_163194137/LConn3 -- T_163194137_400000;150000_Subestação_de_Porto_de_Lagos/RConn3 -- bus129/LConn1
  T_163214309__/RConn1 -- L_163214309/LConn1
  T_163214309__/RConn2 -- L_163214309/LConn2
  L_163214309/LConn3 -- T_163214309__/RConn3 -- bus130/LConn1
  T_144635502_150000_Subestação_de_Ermidas_Sado/RConn1 -- L_144635502/LConn1
  T_144635502_150000_Subestação_de_Ermidas_Sado/RConn2 -- L_144635502/LConn2
  L_144635502/LConn3 -- T_144635502_150000_Subestação_de_Ermidas_Sado/RConn3 -- bus131/LConn1
  T_163214310_150000_/RConn1 -- L_163214310/LConn1
  T_163214310_150000_/RConn2 -- L_163214310/LConn2
  L_163214310/LConn3 -- T_163214310_150000_/RConn3 -- bus132/LConn1
  T_163214308__/RConn1 -- L_163214308/LConn1
  T_163214308__/RConn2 -- L_163214308/LConn2
  L_163214308/LConn3 -- T_163214308__/RConn3 -- bus133/LConn1
  T_163227021_150000;60000_Subestação_de_Trafaria/RConn1 -- L_163227021/LConn1
  T_163227021_150000;60000_Subestação_de_Trafaria/RConn2 -- L_163227021/LConn2
  L_163227021/LConn3 -- T_163227021_150000;60000_Subestação_de_Trafaria/RConn3 -- bus134/LConn1
  T_171253574_150000_/RConn1 -- L_171253574/LConn1
  T_171253574_150000_/RConn2 -- L_171253574/LConn2
  L_171253574/LConn3 -- T_171253574_150000_/RConn3 -- bus135/LConn1
  T_93512590_150000;60000_Subestação_de_Estoi/RConn1 -- L_93512590/LConn1
  T_93512590_150000;60000_Subestação_de_Estoi/RConn2 -- L_93512590/LConn2
  L_93512590/LConn3 -- T_93512590_150000;60000_Subestação_de_Estoi/RConn3 -- bus136/LConn1
  T_201459319_400000;150000_Subestação_REN_Casas_Baixas/RConn1 -- L_201459319/LConn1
  T_201459319_400000;150000_Subestação_REN_Casas_Baixas/RConn2 -- L_201459319/LConn2
  L_201459319/LConn3 -- T_201459319_400000;150000_Subestação_REN_Casas_Baixas/RConn3 -- bus137/LConn1
  T_144711815_150000;60000_Subestação_de_Tunes/RConn1 -- L_144711815/LConn1
  T_144711815_150000;60000_Subestação_de_Tunes/RConn2 -- L_144711815/LConn2
  L_144711815/LConn3 -- T_144711815_150000;60000_Subestação_de_Tunes/RConn3 -- bus138/LConn1
  T_151061905_150000_Subestação_de_Oleiros/RConn1 -- L_151061905/LConn1
  T_151061905_150000_Subestação_de_Oleiros/RConn2 -- L_151061905/LConn2
  L_151061905/LConn3 -- T_151061905_150000_Subestação_de_Oleiros/RConn3 -- bus139/LConn1
  T_151061928_150000;60000_Subestação_de_Vila_Fria/RConn1 -- L_151061928/LConn1
  T_151061928_150000;60000_Subestação_de_Vila_Fria/RConn2 -- L_151061928/LConn2
  L_151061928/LConn3 -- T_151061928_150000;60000_Subestação_de_Vila_Fria/RConn3 -- bus140/LConn1
  T_100898242_150000;60000_Subestação_de_Ermesinde/RConn1 -- L_100898242/LConn1
  T_100898242_150000;60000_Subestação_de_Ermesinde/RConn2 -- L_100898242/LConn2
  L_100898242/LConn3 -- T_100898242_150000;60000_Subestação_de_Ermesinde/RConn3 -- bus141/LConn1
  T_163226990_150000_/RConn1 -- L_163226990/LConn1
  T_163226990_150000_/RConn2 -- L_163226990/LConn2
  L_163226990/LConn3 -- T_163226990_150000_/RConn3 -- bus142/LConn1
  T_151061920_150000_/RConn1 -- L_151061920/LConn1
  T_151061920_150000_/RConn2 -- L_151061920/LConn2
  L_151061920/LConn3 -- T_151061920_150000_/RConn3 -- bus143/LConn1
  T_163226982_150000_Subestação_de_Pegões/RConn1 -- L_163226982/LConn1
  T_163226982_150000_Subestação_de_Pegões/RConn2 -- L_163226982/LConn2
  L_163226982/LConn3 -- T_163226982_150000_Subestação_de_Pegões/RConn3 -- bus144/LConn1
  T_162512815_150000;60000_Subestação_de_Évora/RConn1 -- L_162512815/LConn1
  T_162512815_150000;60000_Subestação_de_Évora/RConn2 -- L_162512815/LConn2
  L_162512815/LConn3 -- T_162512815_150000;60000_Subestação_de_Évora/RConn3 -- bus145/LConn1
  T_151069425_150000_/RConn1 -- L_151069425/LConn1
  T_151069425_150000_/RConn2 -- L_151069425/LConn2
